simulink model "model"  (R2014a)
(part 3 of 4)

  bus249 : powerlib/Measurements/Load Flow Bus  LConnTagsString=a  ID=bus249  Vbase=110000  Vref=1  Vangle=0  VLF=1  angleLF=0
      settings: AttributesFormatString=|
      | %<ID>
      | %<Vbase>V
      | %<VLF>pu
      | %<angleLF>deg.
      | %<Name>
  bus25 : powerlib/Measurements/Load Flow Bus  LConnTagsString=a  ID=bus25  Vbase=110000  Vref=1  Vangle=0  VLF=1  angleLF=0
      settings: AttributesFormatString=|
      | %<ID>
      | %<Vbase>V
      | %<VLF>pu
      | %<angleLF>deg.
      | %<Name>
  bus250 : powerlib/Measurements/Load Flow Bus  LConnTagsString=a  ID=bus250  Vbase=110000  Vref=1  Vangle=0  VLF=1  angleLF=0
      settings: AttributesFormatString=|
      | %<ID>
      | %<Vbase>V
      | %<VLF>pu
      | %<angleLF>deg.
      | %<Name>
  bus251 : powerlib/Measurements/Load Flow Bus  LConnTagsString=a  ID=bus251  Vbase=110000  Vref=1  Vangle=0  VLF=1  angleLF=0
      settings: AttributesFormatString=|
      | %<ID>
      | %<Vbase>V
      | %<VLF>pu
      | %<angleLF>deg.
      | %<Name>
  bus252 : powerlib/Measurements/Load Flow Bus  LConnTagsString=a  ID=bus252  Vbase=110000  Vref=1  Vangle=0  VLF=1  angleLF=0
      settings: AttributesFormatString=|
      | %<ID>
      | %<Vbase>V
      | %<VLF>pu
      | %<angleLF>deg.
      | %<Name>
  bus253 : powerlib/Measurements/Load Flow Bus  LConnTagsString=a  ID=bus253  Vbase=110000  Vref=1  Vangle=0  VLF=1  angleLF=0
      settings: AttributesFormatString=|
      | %<ID>
      | %<Vbase>V
      | %<VLF>pu
      | %<angleLF>deg.
      | %<Name>
  bus254 : powerlib/Measurements/Load Flow Bus  LConnTagsString=a  ID=bus254  Vbase=110000  Vref=1  Vangle=0  VLF=1  angleLF=0
      settings: AttributesFormatString=|
      | %<ID>
      | %<Vbase>V
      | %<VLF>pu
      | %<angleLF>deg.
      | %<Name>
  bus255 : powerlib/Measurements/Load Flow Bus  LConnTagsString=a  ID=bus255  Vbase=110000  Vref=1  Vangle=0  VLF=1  angleLF=0
      settings: AttributesFormatString=|
      | %<ID>
      | %<Vbase>V
      | %<VLF>pu
      | %<angleLF>deg.
      | %<Name>
  bus256 : powerlib/Measurements/Load Flow Bus  LConnTagsString=a  ID=bus256  Vbase=110000  Vref=1  Vangle=0  VLF=1  angleLF=0
      settings: AttributesFormatString=|
      | %<ID>
      | %<Vbase>V
      | %<VLF>pu
      | %<angleLF>deg.
      | %<Name>
  bus257 : powerlib/Measurements/Load Flow Bus  LConnTagsString=a  ID=bus257  Vbase=110000  Vref=1  Vangle=0  VLF=1  angleLF=0
      settings: AttributesFormatString=|
      | %<ID>
      | %<Vbase>V
      | %<VLF>pu
      | %<angleLF>deg.
      | %<Name>
  bus258 : powerlib/Measurements/Load Flow Bus  LConnTagsString=a  ID=bus258  Vbase=110000  Vref=1  Vangle=0  VLF=1  angleLF=0
      settings: AttributesFormatString=|
      | %<ID>
      | %<Vbase>V
      | %<VLF>pu
      | %<angleLF>deg.
      | %<Name>
  bus259 : powerlib/Measurements/Load Flow Bus  LConnTagsString=a  ID=bus259  Vbase=110000  Vref=1  Vangle=0  VLF=1  angleLF=0
      settings: AttributesFormatString=|
      | %<ID>
      | %<Vbase>V
      | %<VLF>pu
      | %<angleLF>deg.
      | %<Name>
  bus26 : powerlib/Measurements/Load Flow Bus  LConnTagsString=a  ID=bus26  Vbase=110000  Vref=1  Vangle=0  VLF=1  angleLF=0
      settings: AttributesFormatString=|
      | %<ID>
      | %<Vbase>V
      | %<VLF>pu
      | %<angleLF>deg.
      | %<Name>
  bus260 : powerlib/Measurements/Load Flow Bus  LConnTagsString=a  ID=bus260  Vbase=110000  Vref=1  Vangle=0  VLF=1  angleLF=0
      settings: AttributesFormatString=|
      | %<ID>
      | %<Vbase>V
      | %<VLF>pu
      | %<angleLF>deg.
      | %<Name>
  bus261 : powerlib/Measurements/Load Flow Bus  LConnTagsString=a  ID=bus261  Vbase=110000  Vref=1  Vangle=0  VLF=1  angleLF=0
      settings: AttributesFormatString=|
      | %<ID>
      | %<Vbase>V
      | %<VLF>pu
      | %<angleLF>deg.
      | %<Name>
  bus262 : powerlib/Measurements/Load Flow Bus  LConnTagsString=a  ID=bus262  Vbase=110000  Vref=1  Vangle=0  VLF=1  angleLF=0
      settings: AttributesFormatString=|
      | %<ID>
      | %<Vbase>V
      | %<VLF>pu
      | %<angleLF>deg.
      | %<Name>
  bus263 : powerlib/Measurements/Load Flow Bus  LConnTagsString=a  ID=bus263  Vbase=110000  Vref=1  Vangle=0  VLF=1  angleLF=0
      settings: AttributesFormatString=|
      | %<ID>
      | %<Vbase>V
      | %<VLF>pu
      | %<angleLF>deg.
      | %<Name>
  bus264 : powerlib/Measurements/Load Flow Bus  LConnTagsString=a  ID=bus264  Vbase=110000  Vref=1  Vangle=0  VLF=1  angleLF=0
      settings: AttributesFormatString=|
      | %<ID>
      | %<Vbase>V
      | %<VLF>pu
      | %<angleLF>deg.
      | %<Name>
  bus265 : powerlib/Measurements/Load Flow Bus  LConnTagsString=a  ID=bus265  Vbase=110000  Vref=1  Vangle=0  VLF=1  angleLF=0
      settings: AttributesFormatString=|
      | %<ID>
      | %<Vbase>V
      | %<VLF>pu
      | %<angleLF>deg.
      | %<Name>
  bus266 : powerlib/Measurements/Load Flow Bus  LConnTagsString=a  ID=bus266  Vbase=110000  Vref=1  Vangle=0  VLF=1  angleLF=0
      settings: AttributesFormatString=|
      | %<ID>
      | %<Vbase>V
      | %<VLF>pu
      | %<angleLF>deg.
      | %<Name>
  bus267 : powerlib/Measurements/Load Flow Bus  LConnTagsString=a  ID=bus267  Vbase=110000  Vref=1  Vangle=0  VLF=1  angleLF=0
      settings: AttributesFormatString=|
      | %<ID>
      | %<Vbase>V
      | %<VLF>pu
      | %<angleLF>deg.
      | %<Name>
  bus268 : powerlib/Measurements/Load Flow Bus  LConnTagsString=a  ID=bus268  Vbase=110000  Vref=1  Vangle=0  VLF=1  angleLF=0
      settings: AttributesFormatString=|
      | %<ID>
      | %<Vbase>V
      | %<VLF>pu
      | %<angleLF>deg.
      | %<Name>
  bus269 : powerlib/Measurements/Load Flow Bus  LConnTagsString=a  ID=bus269  Vbase=110000  Vref=1  Vangle=0  VLF=1  angleLF=0
      settings: AttributesFormatString=|
      | %<ID>
      | %<Vbase>V
      | %<VLF>pu
      | %<angleLF>deg.
      | %<Name>
  bus27 : powerlib/Measurements/Load Flow Bus  LConnTagsString=a  ID=bus27  Vbase=110000  Vref=1  Vangle=0  VLF=1  angleLF=0
      settings: AttributesFormatString=|
      | %<ID>
      | %<Vbase>V
      | %<VLF>pu
      | %<angleLF>deg.
      | %<Name>
  bus270 : powerlib/Measurements/Load Flow Bus  LConnTagsString=a  ID=bus270  Vbase=110000  Vref=1  Vangle=0  VLF=1  angleLF=0
      settings: AttributesFormatString=|
      | %<ID>
      | %<Vbase>V
      | %<VLF>pu
      | %<angleLF>deg.
      | %<Name>
  bus271 : powerlib/Measurements/Load Flow Bus  LConnTagsString=a  ID=bus271  Vbase=110000  Vref=1  Vangle=0  VLF=1  angleLF=0
      settings: AttributesFormatString=|
      | %<ID>
      | %<Vbase>V
      | %<VLF>pu
      | %<angleLF>deg.
      | %<Name>
  bus272 : powerlib/Measurements/Load Flow Bus  LConnTagsString=a  ID=bus272  Vbase=110000  Vref=1  Vangle=0  VLF=1  angleLF=0
      settings: AttributesFormatString=|
      | %<ID>
      | %<Vbase>V
      | %<VLF>pu
      | %<angleLF>deg.
      | %<Name>
  bus273 : powerlib/Measurements/Load Flow Bus  LConnTagsString=a  ID=bus273  Vbase=110000  Vref=1  Vangle=0  VLF=1  angleLF=0
      settings: AttributesFormatString=|
      | %<ID>
      | %<Vbase>V
      | %<VLF>pu
      | %<angleLF>deg.
      | %<Name>
  bus274 : powerlib/Measurements/Load Flow Bus  LConnTagsString=a  ID=bus274  Vbase=110000  Vref=1  Vangle=0  VLF=1  angleLF=0
      settings: AttributesFormatString=|
      | %<ID>
      | %<Vbase>V
      | %<VLF>pu
      | %<angleLF>deg.
      | %<Name>
  bus275 : powerlib/Measurements/Load Flow Bus  LConnTagsString=a  ID=bus275  Vbase=110000  Vref=1  Vangle=0  VLF=1  angleLF=0
      settings: AttributesFormatString=|
      | %<ID>
      | %<Vbase>V
      | %<VLF>pu
      | %<angleLF>deg.
      | %<Name>
  bus276 : powerlib/Measurements/Load Flow Bus  LConnTagsString=a  ID=bus276  Vbase=110000  Vref=1  Vangle=0  VLF=1  angleLF=0
      settings: AttributesFormatString=|
      | %<ID>
      | %<Vbase>V
      | %<VLF>pu
      | %<angleLF>deg.
      | %<Name>
  bus277 : powerlib/Measurements/Load Flow Bus  LConnTagsString=a  ID=bus277  Vbase=110000  Vref=1  Vangle=0  VLF=1  angleLF=0
      settings: AttributesFormatString=|
      | %<ID>
      | %<Vbase>V
      | %<VLF>pu
      | %<angleLF>deg.
      | %<Name>
  bus278 : powerlib/Measurements/Load Flow Bus  LConnTagsString=a  ID=bus278  Vbase=110000  Vref=1  Vangle=0  VLF=1  angleLF=0
      settings: AttributesFormatString=|
      | %<ID>
      | %<Vbase>V
      | %<VLF>pu
      | %<angleLF>deg.
      | %<Name>
  bus279 : powerlib/Measurements/Load Flow Bus  LConnTagsString=a  ID=bus279  Vbase=110000  Vref=1  Vangle=0  VLF=1  angleLF=0
      settings: AttributesFormatString=|
      | %<ID>
      | %<Vbase>V
      | %<VLF>pu
      | %<angleLF>deg.
      | %<Name>
  bus28 : powerlib/Measurements/Load Flow Bus  LConnTagsString=a  ID=bus28  Vbase=110000  Vref=1  Vangle=0  VLF=1  angleLF=0
      settings: AttributesFormatString=|
      | %<ID>
      | %<Vbase>V
      | %<VLF>pu
      | %<angleLF>deg.
      | %<Name>
  bus280 : powerlib/Measurements/Load Flow Bus  LConnTagsString=a  ID=bus280  Vbase=110000  Vref=1  Vangle=0  VLF=1  angleLF=0
      settings: AttributesFormatString=|
      | %<ID>
      | %<Vbase>V
      | %<VLF>pu
      | %<angleLF>deg.
      | %<Name>
  bus281 : powerlib/Measurements/Load Flow Bus  LConnTagsString=a  ID=bus281  Vbase=110000  Vref=1  Vangle=0  VLF=1  angleLF=0
      settings: AttributesFormatString=|
      | %<ID>
      | %<Vbase>V
      | %<VLF>pu
      | %<angleLF>deg.
      | %<Name>
  bus282 : powerlib/Measurements/Load Flow Bus  LConnTagsString=a  ID=bus282  Vbase=110000  Vref=1  Vangle=0  VLF=1  angleLF=0
      settings: AttributesFormatString=|
      | %<ID>
      | %<Vbase>V
      | %<VLF>pu
      | %<angleLF>deg.
      | %<Name>
  bus283 : powerlib/Measurements/Load Flow Bus  LConnTagsString=a  ID=bus283  Vbase=110000  Vref=1  Vangle=0  VLF=1  angleLF=0
      settings: AttributesFormatString=|
      | %<ID>
      | %<Vbase>V
      | %<VLF>pu
      | %<angleLF>deg.
      | %<Name>
  bus284 : powerlib/Measurements/Load Flow Bus  LConnTagsString=a  ID=bus284  Vbase=110000  Vref=1  Vangle=0  VLF=1  angleLF=0
      settings: AttributesFormatString=|
      | %<ID>
      | %<Vbase>V
      | %<VLF>pu
      | %<angleLF>deg.
      | %<Name>
  bus285 : powerlib/Measurements/Load Flow Bus  LConnTagsString=a  ID=bus285  Vbase=110000  Vref=1  Vangle=0  VLF=1  angleLF=0
      settings: AttributesFormatString=|
      | %<ID>
      | %<Vbase>V
      | %<VLF>pu
      | %<angleLF>deg.
      | %<Name>
  bus286 : powerlib/Measurements/Load Flow Bus  LConnTagsString=a  ID=bus286  Vbase=110000  Vref=1  Vangle=0  VLF=1  angleLF=0
      settings: AttributesFormatString=|
      | %<ID>
      | %<Vbase>V
      | %<VLF>pu
      | %<angleLF>deg.
      | %<Name>
  bus287 : powerlib/Measurements/Load Flow Bus  LConnTagsString=a  ID=bus287  Vbase=110000  Vref=1  Vangle=0  VLF=1  angleLF=0
      settings: AttributesFormatString=|
      | %<ID>
      | %<Vbase>V
      | %<VLF>pu
      | %<angleLF>deg.
      | %<Name>
  bus288 : powerlib/Measurements/Load Flow Bus  LConnTagsString=a  ID=bus288  Vbase=110000  Vref=1  Vangle=0  VLF=1  angleLF=0
      settings: AttributesFormatString=|
      | %<ID>
      | %<Vbase>V
      | %<VLF>pu
      | %<angleLF>deg.
      | %<Name>
  bus289 : powerlib/Measurements/Load Flow Bus  LConnTagsString=a  ID=bus289  Vbase=110000  Vref=1  Vangle=0  VLF=1  angleLF=0
      settings: AttributesFormatString=|
      | %<ID>
      | %<Vbase>V
      | %<VLF>pu
      | %<angleLF>deg.
      | %<Name>
  bus29 : powerlib/Measurements/Load Flow Bus  LConnTagsString=a  ID=bus29  Vbase=110000  Vref=1  Vangle=0  VLF=1  angleLF=0
      settings: AttributesFormatString=|
      | %<ID>
      | %<Vbase>V
      | %<VLF>pu
      | %<angleLF>deg.
      | %<Name>
  bus290 : powerlib/Measurements/Load Flow Bus  LConnTagsString=a  ID=bus290  Vbase=110000  Vref=1  Vangle=0  VLF=1  angleLF=0
      settings: AttributesFormatString=|
      | %<ID>
      | %<Vbase>V
      | %<VLF>pu
      | %<angleLF>deg.
      | %<Name>
  bus291 : powerlib/Measurements/Load Flow Bus  LConnTagsString=a  ID=bus291  Vbase=110000  Vref=1  Vangle=0  VLF=1  angleLF=0
      settings: AttributesFormatString=|
      | %<ID>
      | %<Vbase>V
      | %<VLF>pu
      | %<angleLF>deg.
      | %<Name>
  bus292 : powerlib/Measurements/Load Flow Bus  LConnTagsString=a  ID=bus292  Vbase=110000  Vref=1  Vangle=0  VLF=1  angleLF=0
      settings: AttributesFormatString=|
      | %<ID>
      | %<Vbase>V
      | %<VLF>pu
      | %<angleLF>deg.
      | %<Name>
  bus293 : powerlib/Measurements/Load Flow Bus  LConnTagsString=a  ID=bus293  Vbase=110000  Vref=1  Vangle=0  VLF=1  angleLF=0
      settings: AttributesFormatString=|
      | %<ID>
      | %<Vbase>V
      | %<VLF>pu
      | %<angleLF>deg.
      | %<Name>
  bus294 : powerlib/Measurements/Load Flow Bus  LConnTagsString=a  ID=bus294  Vbase=110000  Vref=1  Vangle=0  VLF=1  angleLF=0
      settings: AttributesFormatString=|
      | %<ID>
      | %<Vbase>V
      | %<VLF>pu
      | %<angleLF>deg.
      | %<Name>
  bus295 : powerlib/Measurements/Load Flow Bus  LConnTagsString=a  ID=bus295  Vbase=110000  Vref=1  Vangle=0  VLF=1  angleLF=0
      settings: AttributesFormatString=|
      | %<ID>
      | %<Vbase>V
      | %<VLF>pu
      | %<angleLF>deg.
      | %<Name>
  bus296 : powerlib/Measurements/Load Flow Bus  LConnTagsString=a  ID=bus296  Vbase=110000  Vref=1  Vangle=0  VLF=1  angleLF=0
      settings: AttributesFormatString=|
      | %<ID>
      | %<Vbase>V
      | %<VLF>pu
      | %<angleLF>deg.
      | %<Name>
  bus297 : powerlib/Measurements/Load Flow Bus  LConnTagsString=a  ID=bus297  Vbase=110000  Vref=1  Vangle=0  VLF=1  angleLF=0
      settings: AttributesFormatString=|
      | %<ID>
      | %<Vbase>V
      | %<VLF>pu
      | %<angleLF>deg.
      | %<Name>
  bus298 : powerlib/Measurements/Load Flow Bus  LConnTagsString=a  ID=bus298  Vbase=110000  Vref=1  Vangle=0  VLF=1  angleLF=0
      settings: AttributesFormatString=|
      | %<ID>
      | %<Vbase>V
      | %<VLF>pu
      | %<angleLF>deg.
      | %<Name>
  bus299 : powerlib/Measurements/Load Flow Bus  LConnTagsString=a  ID=bus299  Vbase=110000  Vref=1  Vangle=0  VLF=1  angleLF=0
      settings: AttributesFormatString=|
      | %<ID>
      | %<Vbase>V
      | %<VLF>pu
      | %<angleLF>deg.
      | %<Name>
  bus3 : powerlib/Measurements/Load Flow Bus  LConnTagsString=a  ID=bus3  Vbase=110000  Vref=1  Vangle=0  VLF=1  angleLF=0
      settings: AttributesFormatString=|
      | %<ID>
      | %<Vbase>V
      | %<VLF>pu
      | %<angleLF>deg.
      | %<Name>
  bus30 : powerlib/Measurements/Load Flow Bus  LConnTagsString=a  ID=bus30  Vbase=110000  Vref=1  Vangle=0  VLF=1  angleLF=0
      settings: AttributesFormatString=|
      | %<ID>
      | %<Vbase>V
      | %<VLF>pu
      | %<angleLF>deg.
      | %<Name>
  bus300 : powerlib/Measurements/Load Flow Bus  LConnTagsString=a  ID=bus300  Vbase=110000  Vref=1  Vangle=0  VLF=1  angleLF=0
      settings: AttributesFormatString=|
      | %<ID>
      | %<Vbase>V
      | %<VLF>pu
      | %<angleLF>deg.
      | %<Name>
  bus301 : powerlib/Measurements/Load Flow Bus  LConnTagsString=a  ID=bus301  Vbase=110000  Vref=1  Vangle=0  VLF=1  angleLF=0
      settings: AttributesFormatString=|
      | %<ID>
      | %<Vbase>V
      | %<VLF>pu
      | %<angleLF>deg.
      | %<Name>
  bus302 : powerlib/Measurements/Load Flow Bus  LConnTagsString=a  ID=bus302  Vbase=110000  Vref=1  Vangle=0  VLF=1  angleLF=0
      settings: AttributesFormatString=|
      | %<ID>
      | %<Vbase>V
      | %<VLF>pu
      | %<angleLF>deg.
      | %<Name>
  bus303 : powerlib/Measurements/Load Flow Bus  LConnTagsString=a  ID=bus303  Vbase=110000  Vref=1  Vangle=0  VLF=1  angleLF=0
      settings: AttributesFormatString=|
      | %<ID>
      | %<Vbase>V
      | %<VLF>pu
      | %<angleLF>deg.
      | %<Name>
  bus304 : powerlib/Measurements/Load Flow Bus  LConnTagsString=a  ID=bus304  Vbase=110000  Vref=1  Vangle=0  VLF=1  angleLF=0
      settings: AttributesFormatString=|
      | %<ID>
      | %<Vbase>V
      | %<VLF>pu
      | %<angleLF>deg.
      | %<Name>
  bus305 : powerlib/Measurements/Load Flow Bus  LConnTagsString=a  ID=bus305  Vbase=110000  Vref=1  Vangle=0  VLF=1  angleLF=0
      settings: AttributesFormatString=|
      | %<ID>
      | %<Vbase>V
      | %<VLF>pu
      | %<angleLF>deg.
      | %<Name>
  bus306 : powerlib/Measurements/Load Flow Bus  LConnTagsString=a  ID=bus306  Vbase=110000  Vref=1  Vangle=0  VLF=1  angleLF=0
      settings: AttributesFormatString=|
      | %<ID>
      | %<Vbase>V
      | %<VLF>pu
      | %<angleLF>deg.
      | %<Name>
  bus307 : powerlib/Measurements/Load Flow Bus  LConnTagsString=a  ID=bus307  Vbase=110000  Vref=1  Vangle=0  VLF=1  angleLF=0
      settings: AttributesFormatString=|
      | %<ID>
      | %<Vbase>V
      | %<VLF>pu
      | %<angleLF>deg.
      | %<Name>
  bus308 : powerlib/Measurements/Load Flow Bus  LConnTagsString=a  ID=bus308  Vbase=110000  Vref=1  Vangle=0  VLF=1  angleLF=0
      settings: AttributesFormatString=|
      | %<ID>
      | %<Vbase>V
      | %<VLF>pu
      | %<angleLF>deg.
      | %<Name>
  bus309 : powerlib/Measurements/Load Flow Bus  LConnTagsString=a  ID=bus309  Vbase=110000  Vref=1  Vangle=0  VLF=1  angleLF=0
      settings: AttributesFormatString=|
      | %<ID>
      | %<Vbase>V
      | %<VLF>pu
      | %<angleLF>deg.
      | %<Name>
  bus31 : powerlib/Measurements/Load Flow Bus  LConnTagsString=a  ID=bus31  Vbase=110000  Vref=1  Vangle=0  VLF=1  angleLF=0
      settings: AttributesFormatString=|
      | %<ID>
      | %<Vbase>V
      | %<VLF>pu
      | %<angleLF>deg.
      | %<Name>
  bus310 : powerlib/Measurements/Load Flow Bus  LConnTagsString=a  ID=bus310  Vbase=110000  Vref=1  Vangle=0  VLF=1  angleLF=0
      settings: AttributesFormatString=|
      | %<ID>
      | %<Vbase>V
      | %<VLF>pu
      | %<angleLF>deg.
      | %<Name>
  bus311 : powerlib/Measurements/Load Flow Bus  LConnTagsString=a  ID=bus311  Vbase=110000  Vref=1  Vangle=0  VLF=1  angleLF=0
      settings: AttributesFormatString=|
      | %<ID>
      | %<Vbase>V
      | %<VLF>pu
      | %<angleLF>deg.
      | %<Name>
  bus312 : powerlib/Measurements/Load Flow Bus  LConnTagsString=a  ID=bus312  Vbase=110000  Vref=1  Vangle=0  VLF=1  angleLF=0
      settings: AttributesFormatString=|
      | %<ID>
      | %<Vbase>V
      | %<VLF>pu
      | %<angleLF>deg.
      | %<Name>
  bus313 : powerlib/Measurements/Load Flow Bus  LConnTagsString=a  ID=bus313  Vbase=110000  Vref=1  Vangle=0  VLF=1  angleLF=0
      settings: AttributesFormatString=|
      | %<ID>
      | %<Vbase>V
      | %<VLF>pu
      | %<angleLF>deg.
      | %<Name>
  bus314 : powerlib/Measurements/Load Flow Bus  LConnTagsString=a  ID=bus314  Vbase=110000  Vref=1  Vangle=0  VLF=1  angleLF=0
      settings: AttributesFormatString=|
      | %<ID>
      | %<Vbase>V
      | %<VLF>pu
      | %<angleLF>deg.
      | %<Name>
  bus315 : powerlib/Measurements/Load Flow Bus  LConnTagsString=a  ID=bus315  Vbase=110000  Vref=1  Vangle=0  VLF=1  angleLF=0
      settings: AttributesFormatString=|
      | %<ID>
      | %<Vbase>V
      | %<VLF>pu
      | %<angleLF>deg.
      | %<Name>
  bus316 : powerlib/Measurements/Load Flow Bus  LConnTagsString=a  ID=bus316  Vbase=110000  Vref=1  Vangle=0  VLF=1  angleLF=0
      settings: AttributesFormatString=|
      | %<ID>
      | %<Vbase>V
      | %<VLF>pu
      | %<angleLF>deg.
      | %<Name>
  bus317 : powerlib/Measurements/Load Flow Bus  LConnTagsString=a  ID=bus317  Vbase=110000  Vref=1  Vangle=0  VLF=1  angleLF=0
      settings: AttributesFormatString=|
      | %<ID>
      | %<Vbase>V
      | %<VLF>pu
      | %<angleLF>deg.
      | %<Name>
  bus318 : powerlib/Measurements/Load Flow Bus  LConnTagsString=a  ID=bus318  Vbase=110000  Vref=1  Vangle=0  VLF=1  angleLF=0
      settings: AttributesFormatString=|
      | %<ID>
      | %<Vbase>V
      | %<VLF>pu
      | %<angleLF>deg.
      | %<Name>
  bus319 : powerlib/Measurements/Load Flow Bus  LConnTagsString=a  ID=bus319  Vbase=110000  Vref=1  Vangle=0  VLF=1  angleLF=0
      settings: AttributesFormatString=|
      | %<ID>
      | %<Vbase>V
      | %<VLF>pu
      | %<angleLF>deg.
      | %<Name>
  bus32 : powerlib/Measurements/Load Flow Bus  LConnTagsString=a  ID=bus32  Vbase=110000  Vref=1  Vangle=0  VLF=1  angleLF=0
      settings: AttributesFormatString=|
      | %<ID>
      | %<Vbase>V
      | %<VLF>pu
      | %<angleLF>deg.
      | %<Name>
  bus320 : powerlib/Measurements/Load Flow Bus  LConnTagsString=a  ID=bus320  Vbase=110000  Vref=1  Vangle=0  VLF=1  angleLF=0
      settings: AttributesFormatString=|
      | %<ID>
      | %<Vbase>V
      | %<VLF>pu
      | %<angleLF>deg.
      | %<Name>
  bus321 : powerlib/Measurements/Load Flow Bus  LConnTagsString=a  ID=bus321  Vbase=110000  Vref=1  Vangle=0  VLF=1  angleLF=0
      settings: AttributesFormatString=|
      | %<ID>
      | %<Vbase>V
      | %<VLF>pu
      | %<angleLF>deg.
      | %<Name>
  bus322 : powerlib/Measurements/Load Flow Bus  LConnTagsString=a  ID=bus322  Vbase=110000  Vref=1  Vangle=0  VLF=1  angleLF=0
      settings: AttributesFormatString=|
      | %<ID>
      | %<Vbase>V
      | %<VLF>pu
      | %<angleLF>deg.
      | %<Name>
  bus323 : powerlib/Measurements/Load Flow Bus  LConnTagsString=a  ID=bus323  Vbase=110000  Vref=1  Vangle=0  VLF=1  angleLF=0
      settings: AttributesFormatString=|
      | %<ID>
      | %<Vbase>V
      | %<VLF>pu
      | %<angleLF>deg.
      | %<Name>
  bus324 : powerlib/Measurements/Load Flow Bus  LConnTagsString=a  ID=bus324  Vbase=110000  Vref=1  Vangle=0  VLF=1  angleLF=0
      settings: AttributesFormatString=|
      | %<ID>
      | %<Vbase>V
      | %<VLF>pu
      | %<angleLF>deg.
      | %<Name>
  bus325 : powerlib/Measurements/Load Flow Bus  LConnTagsString=a  ID=bus325  Vbase=110000  Vref=1  Vangle=0  VLF=1  angleLF=0
      settings: AttributesFormatString=|
      | %<ID>
      | %<Vbase>V
      | %<VLF>pu
      | %<angleLF>deg.
      | %<Name>
  bus326 : powerlib/Measurements/Load Flow Bus  LConnTagsString=a  ID=bus326  Vbase=110000  Vref=1  Vangle=0  VLF=1  angleLF=0
      settings: AttributesFormatString=|
      | %<ID>
      | %<Vbase>V
      | %<VLF>pu
      | %<angleLF>deg.
      | %<Name>
  bus327 : powerlib/Measurements/Load Flow Bus  LConnTagsString=a  ID=bus327  Vbase=110000  Vref=1  Vangle=0  VLF=1  angleLF=0
      settings: AttributesFormatString=|
      | %<ID>
      | %<Vbase>V
      | %<VLF>pu
      | %<angleLF>deg.
      | %<Name>
  bus328 : powerlib/Measurements/Load Flow Bus  LConnTagsString=a  ID=bus328  Vbase=110000  Vref=1  Vangle=0  VLF=1  angleLF=0
      settings: AttributesFormatString=|
      | %<ID>
      | %<Vbase>V
      | %<VLF>pu
      | %<angleLF>deg.
      | %<Name>
  bus329 : powerlib/Measurements/Load Flow Bus  LConnTagsString=a  ID=bus329  Vbase=110000  Vref=1  Vangle=0  VLF=1  angleLF=0
      settings: AttributesFormatString=|
      | %<ID>
      | %<Vbase>V
      | %<VLF>pu
      | %<angleLF>deg.
      | %<Name>
  bus33 : powerlib/Measurements/Load Flow Bus  LConnTagsString=a  ID=bus33  Vbase=110000  Vref=1  Vangle=0  VLF=1  angleLF=0
      settings: AttributesFormatString=|
      | %<ID>
      | %<Vbase>V
      | %<VLF>pu
      | %<angleLF>deg.
      | %<Name>
  bus330 : powerlib/Measurements/Load Flow Bus  LConnTagsString=a  ID=bus330  Vbase=110000  Vref=1  Vangle=0  VLF=1  angleLF=0
      settings: AttributesFormatString=|
      | %<ID>
      | %<Vbase>V
      | %<VLF>pu
      | %<angleLF>deg.
      | %<Name>
  bus331 : powerlib/Measurements/Load Flow Bus  LConnTagsString=a  ID=bus331  Vbase=110000  Vref=1  Vangle=0  VLF=1  angleLF=0
      settings: AttributesFormatString=|
      | %<ID>
      | %<Vbase>V
      | %<VLF>pu
      | %<angleLF>deg.
      | %<Name>
  bus332 : powerlib/Measurements/Load Flow Bus  LConnTagsString=a  ID=bus332  Vbase=110000  Vref=1  Vangle=0  VLF=1  angleLF=0
      settings: AttributesFormatString=|
      | %<ID>
      | %<Vbase>V
      | %<VLF>pu
      | %<angleLF>deg.
      | %<Name>
  bus333 : powerlib/Measurements/Load Flow Bus  LConnTagsString=a  ID=bus333  Vbase=110000  Vref=1  Vangle=0  VLF=1  angleLF=0
      settings: AttributesFormatString=|
      | %<ID>
      | %<Vbase>V
      | %<VLF>pu
      | %<angleLF>deg.
      | %<Name>
  bus334 : powerlib/Measurements/Load Flow Bus  LConnTagsString=a  ID=bus334  Vbase=110000  Vref=1  Vangle=0  VLF=1  angleLF=0
      settings: AttributesFormatString=|
      | %<ID>
      | %<Vbase>V
      | %<VLF>pu
      | %<angleLF>deg.
      | %<Name>
  bus335 : powerlib/Measurements/Load Flow Bus  LConnTagsString=a  ID=bus335  Vbase=110000  Vref=1  Vangle=0  VLF=1  angleLF=0
      settings: AttributesFormatString=|
      | %<ID>
      | %<Vbase>V
      | %<VLF>pu
      | %<angleLF>deg.
      | %<Name>
  bus336 : powerlib/Measurements/Load Flow Bus  LConnTagsString=a  ID=bus336  Vbase=110000  Vref=1  Vangle=0  VLF=1  angleLF=0
      settings: AttributesFormatString=|
      | %<ID>
      | %<Vbase>V
      | %<VLF>pu
      | %<angleLF>deg.
      | %<Name>
  bus337 : powerlib/Measurements/Load Flow Bus  LConnTagsString=a  ID=bus337  Vbase=110000  Vref=1  Vangle=0  VLF=1  angleLF=0
      settings: AttributesFormatString=|
      | %<ID>
      | %<Vbase>V
      | %<VLF>pu
      | %<angleLF>deg.
      | %<Name>
  bus338 : powerlib/Measurements/Load Flow Bus  LConnTagsString=a  ID=bus338  Vbase=110000  Vref=1  Vangle=0  VLF=1  angleLF=0
      settings: AttributesFormatString=|
      | %<ID>
      | %<Vbase>V
      | %<VLF>pu
      | %<angleLF>deg.
      | %<Name>
  bus339 : powerlib/Measurements/Load Flow Bus  LConnTagsString=a  ID=bus339  Vbase=110000  Vref=1  Vangle=0  VLF=1  angleLF=0
      settings: AttributesFormatString=|
      | %<ID>
      | %<Vbase>V
      | %<VLF>pu
      | %<angleLF>deg.
      | %<Name>
  bus34 : powerlib/Measurements/Load Flow Bus  LConnTagsString=a  ID=bus34  Vbase=110000  Vref=1  Vangle=0  VLF=1  angleLF=0
      settings: AttributesFormatString=|
      | %<ID>
      | %<Vbase>V
      | %<VLF>pu
      | %<angleLF>deg.
      | %<Name>
  bus340 : powerlib/Measurements/Load Flow Bus  LConnTagsString=a  ID=bus340  Vbase=110000  Vref=1  Vangle=0  VLF=1  angleLF=0
      settings: AttributesFormatString=|
      | %<ID>
      | %<Vbase>V
      | %<VLF>pu
      | %<angleLF>deg.
      | %<Name>
  bus341 : powerlib/Measurements/Load Flow Bus  LConnTagsString=a  ID=bus341  Vbase=110000  Vref=1  Vangle=0  VLF=1  angleLF=0
      settings: AttributesFormatString=|
      | %<ID>
      | %<Vbase>V
      | %<VLF>pu
      | %<angleLF>deg.
      | %<Name>
  bus342 : powerlib/Measurements/Load Flow Bus  LConnTagsString=a  ID=bus342  Vbase=110000  Vref=1  Vangle=0  VLF=1  angleLF=0
      settings: AttributesFormatString=|
      | %<ID>
      | %<Vbase>V
      | %<VLF>pu
      | %<angleLF>deg.
      | %<Name>
  bus343 : powerlib/Measurements/Load Flow Bus  LConnTagsString=a  ID=bus343  Vbase=110000  Vref=1  Vangle=0  VLF=1  angleLF=0
      settings: AttributesFormatString=|
      | %<ID>
      | %<Vbase>V
      | %<VLF>pu
      | %<angleLF>deg.
      | %<Name>
  bus344 : powerlib/Measurements/Load Flow Bus  LConnTagsString=a  ID=bus344  Vbase=110000  Vref=1  Vangle=0  VLF=1  angleLF=0
      settings: AttributesFormatString=|
      | %<ID>
      | %<Vbase>V
      | %<VLF>pu
      | %<angleLF>deg.
      | %<Name>
  bus345 : powerlib/Measurements/Load Flow Bus  LConnTagsString=a  ID=bus345  Vbase=110000  Vref=1  Vangle=0  VLF=1  angleLF=0
      settings: AttributesFormatString=|
      | %<ID>
      | %<Vbase>V
      | %<VLF>pu
      | %<angleLF>deg.
      | %<Name>
  bus346 : powerlib/Measurements/Load Flow Bus  LConnTagsString=a  ID=bus346  Vbase=110000  Vref=1  Vangle=0  VLF=1  angleLF=0
      settings: AttributesFormatString=|
      | %<ID>
      | %<Vbase>V
      | %<VLF>pu
      | %<angleLF>deg.
      | %<Name>
  bus347 : powerlib/Measurements/Load Flow Bus  LConnTagsString=a  ID=bus347  Vbase=110000  Vref=1  Vangle=0  VLF=1  angleLF=0
      settings: AttributesFormatString=|
      | %<ID>
      | %<Vbase>V
      | %<VLF>pu
      | %<angleLF>deg.
      | %<Name>
  bus348 : powerlib/Measurements/Load Flow Bus  LConnTagsString=a  ID=bus348  Vbase=110000  Vref=1  Vangle=0  VLF=1  angleLF=0
      settings: AttributesFormatString=|
      | %<ID>
      | %<Vbase>V
      | %<VLF>pu
      | %<angleLF>deg.
      | %<Name>
  bus349 : powerlib/Measurements/Load Flow Bus  LConnTagsString=a  ID=bus349  Vbase=110000  Vref=1  Vangle=0  VLF=1  angleLF=0
      settings: AttributesFormatString=|
      | %<ID>
      | %<Vbase>V
      | %<VLF>pu
      | %<angleLF>deg.
      | %<Name>
  bus35 : powerlib/Measurements/Load Flow Bus  LConnTagsString=a  ID=bus35  Vbase=110000  Vref=1  Vangle=0  VLF=1  angleLF=0
      settings: AttributesFormatString=|
      | %<ID>
      | %<Vbase>V
      | %<VLF>pu
      | %<angleLF>deg.
      | %<Name>
  bus350 : powerlib/Measurements/Load Flow Bus  LConnTagsString=a  ID=bus350  Vbase=110000  Vref=1  Vangle=0  VLF=1  angleLF=0
      settings: AttributesFormatString=|
      | %<ID>
      | %<Vbase>V
      | %<VLF>pu
      | %<angleLF>deg.
      | %<Name>
  bus351 : powerlib/Measurements/Load Flow Bus  LConnTagsString=a  ID=bus351  Vbase=110000  Vref=1  Vangle=0  VLF=1  angleLF=0
      settings: AttributesFormatString=|
      | %<ID>
      | %<Vbase>V
      | %<VLF>pu
      | %<angleLF>deg.
      | %<Name>
  bus352 : powerlib/Measurements/Load Flow Bus  LConnTagsString=a  ID=bus352  Vbase=110000  Vref=1  Vangle=0  VLF=1  angleLF=0
      settings: AttributesFormatString=|
      | %<ID>
      | %<Vbase>V
      | %<VLF>pu
      | %<angleLF>deg.
      | %<Name>
  bus353 : powerlib/Measurements/Load Flow Bus  LConnTagsString=a  ID=bus353  Vbase=110000  Vref=1  Vangle=0  VLF=1  angleLF=0
      settings: AttributesFormatString=|
      | %<ID>
      | %<Vbase>V
      | %<VLF>pu
      | %<angleLF>deg.
      | %<Name>
  bus354 : powerlib/Measurements/Load Flow Bus  LConnTagsString=a  ID=bus354  Vbase=110000  Vref=1  Vangle=0  VLF=1  angleLF=0
      settings: AttributesFormatString=|
      | %<ID>
      | %<Vbase>V
      | %<VLF>pu
      | %<angleLF>deg.
      | %<Name>
  bus355 : powerlib/Measurements/Load Flow Bus  LConnTagsString=a  ID=bus355  Vbase=110000  Vref=1  Vangle=0  VLF=1  angleLF=0
      settings: AttributesFormatString=|
      | %<ID>
      | %<Vbase>V
      | %<VLF>pu
      | %<angleLF>deg.
      | %<Name>
  bus356 : powerlib/Measurements/Load Flow Bus  LConnTagsString=a  ID=bus356  Vbase=110000  Vref=1  Vangle=0  VLF=1  angleLF=0
      settings: AttributesFormatString=|
      | %<ID>
      | %<Vbase>V
      | %<VLF>pu
      | %<angleLF>deg.
      | %<Name>
  bus357 : powerlib/Measurements/Load Flow Bus  LConnTagsString=a  ID=bus357  Vbase=110000  Vref=1  Vangle=0  VLF=1  angleLF=0
      settings: AttributesFormatString=|
      | %<ID>
      | %<Vbase>V
      | %<VLF>pu
      | %<angleLF>deg.
      | %<Name>
  bus358 : powerlib/Measurements/Load Flow Bus  LConnTagsString=a  ID=bus358  Vbase=110000  Vref=1  Vangle=0  VLF=1  angleLF=0
      settings: AttributesFormatString=|
      | %<ID>
      | %<Vbase>V
      | %<VLF>pu
      | %<angleLF>deg.
      | %<Name>
  bus359 : powerlib/Measurements/Load Flow Bus  LConnTagsString=a  ID=bus359  Vbase=110000  Vref=1  Vangle=0  VLF=1  angleLF=0
      settings: AttributesFormatString=|
      | %<ID>
      | %<Vbase>V
      | %<VLF>pu
      | %<angleLF>deg.
      | %<Name>
  bus36 : powerlib/Measurements/Load Flow Bus  LConnTagsString=a  ID=bus36  Vbase=110000  Vref=1  Vangle=0  VLF=1  angleLF=0
      settings: AttributesFormatString=|
      | %<ID>
      | %<Vbase>V
      | %<VLF>pu
      | %<angleLF>deg.
      | %<Name>
  bus360 : powerlib/Measurements/Load Flow Bus  LConnTagsString=a  ID=bus360  Vbase=110000  Vref=1  Vangle=0  VLF=1  angleLF=0
      settings: AttributesFormatString=|
      | %<ID>
      | %<Vbase>V
      | %<VLF>pu
      | %<angleLF>deg.
      | %<Name>
  bus361 : powerlib/Measurements/Load Flow Bus  LConnTagsString=a  ID=bus361  Vbase=110000  Vref=1  Vangle=0  VLF=1  angleLF=0
      settings: AttributesFormatString=|
      | %<ID>
      | %<Vbase>V
      | %<VLF>pu
      | %<angleLF>deg.
      | %<Name>
  bus362 : powerlib/Measurements/Load Flow Bus  LConnTagsString=a  ID=bus362  Vbase=110000  Vref=1  Vangle=0  VLF=1  angleLF=0
      settings: AttributesFormatString=|
      | %<ID>
      | %<Vbase>V
      | %<VLF>pu
      | %<angleLF>deg.
      | %<Name>
  bus363 : powerlib/Measurements/Load Flow Bus  LConnTagsString=a  ID=bus363  Vbase=110000  Vref=1  Vangle=0  VLF=1  angleLF=0
      settings: AttributesFormatString=|
      | %<ID>
      | %<Vbase>V
      | %<VLF>pu
      | %<angleLF>deg.
      | %<Name>
  bus364 : powerlib/Measurements/Load Flow Bus  LConnTagsString=a  ID=bus364  Vbase=110000  Vref=1  Vangle=0  VLF=1  angleLF=0
      settings: AttributesFormatString=|
      | %<ID>
      | %<Vbase>V
      | %<VLF>pu
      | %<angleLF>deg.
      | %<Name>
  bus365 : powerlib/Measurements/Load Flow Bus  LConnTagsString=a  ID=bus365  Vbase=110000  Vref=1  Vangle=0  VLF=1  angleLF=0
      settings: AttributesFormatString=|
      | %<ID>
      | %<Vbase>V
      | %<VLF>pu
      | %<angleLF>deg.
      | %<Name>
  bus366 : powerlib/Measurements/Load Flow Bus  LConnTagsString=a  ID=bus366  Vbase=110000  Vref=1  Vangle=0  VLF=1  angleLF=0
      settings: AttributesFormatString=|
      | %<ID>
      | %<Vbase>V
      | %<VLF>pu
      | %<angleLF>deg.
      | %<Name>
  bus367 : powerlib/Measurements/Load Flow Bus  LConnTagsString=a  ID=bus367  Vbase=110000  Vref=1  Vangle=0  VLF=1  angleLF=0
      settings: AttributesFormatString=|
      | %<ID>
      | %<Vbase>V
      | %<VLF>pu
      | %<angleLF>deg.
      | %<Name>
  bus368 : powerlib/Measurements/Load Flow Bus  LConnTagsString=a  ID=bus368  Vbase=110000  Vref=1  Vangle=0  VLF=1  angleLF=0
      settings: AttributesFormatString=|
      | %<ID>
      | %<Vbase>V
      | %<VLF>pu
      | %<angleLF>deg.
      | %<Name>
  bus369 : powerlib/Measurements/Load Flow Bus  LConnTagsString=a  ID=bus369  Vbase=110000  Vref=1  Vangle=0  VLF=1  angleLF=0
      settings: AttributesFormatString=|
      | %<ID>
      | %<Vbase>V
      | %<VLF>pu
      | %<angleLF>deg.
      | %<Name>
  bus37 : powerlib/Measurements/Load Flow Bus  LConnTagsString=a  ID=bus37  Vbase=110000  Vref=1  Vangle=0  VLF=1  angleLF=0
      settings: AttributesFormatString=|
      | %<ID>
      | %<Vbase>V
      | %<VLF>pu
      | %<angleLF>deg.
      | %<Name>
  bus370 : powerlib/Measurements/Load Flow Bus  LConnTagsString=a  ID=bus370  Vbase=110000  Vref=1  Vangle=0  VLF=1  angleLF=0
      settings: AttributesFormatString=|
      | %<ID>
      | %<Vbase>V
      | %<VLF>pu
      | %<angleLF>deg.
      | %<Name>
  bus371 : powerlib/Measurements/Load Flow Bus  LConnTagsString=a  ID=bus371  Vbase=110000  Vref=1  Vangle=0  VLF=1  angleLF=0
      settings: AttributesFormatString=|
      | %<ID>
      | %<Vbase>V
      | %<VLF>pu
      | %<angleLF>deg.
      | %<Name>
  bus372 : powerlib/Measurements/Load Flow Bus  LConnTagsString=a  ID=bus372  Vbase=330000  Vref=1  Vangle=0  VLF=1  angleLF=0
      settings: AttributesFormatString=|
      | %<ID>
      | %<Vbase>V
      | %<VLF>pu
      | %<angleLF>deg.
      | %<Name>
  bus373 : powerlib/Measurements/Load Flow Bus  LConnTagsString=a  ID=bus373  Vbase=330000  Vref=1  Vangle=0  VLF=1  angleLF=0
      settings: AttributesFormatString=|
      | %<ID>
      | %<Vbase>V
      | %<VLF>pu
      | %<angleLF>deg.
      | %<Name>
  bus374 : powerlib/Measurements/Load Flow Bus  LConnTagsString=a  ID=bus374  Vbase=330000  Vref=1  Vangle=0  VLF=1  angleLF=0
      settings: AttributesFormatString=|
      | %<ID>
      | %<Vbase>V
      | %<VLF>pu
      | %<angleLF>deg.
      | %<Name>
  bus375 : powerlib/Measurements/Load Flow Bus  LConnTagsString=a  ID=bus375  Vbase=330000  Vref=1  Vangle=0  VLF=1  angleLF=0
      settings: AttributesFormatString=|
      | %<ID>
      | %<Vbase>V
      | %<VLF>pu
      | %<angleLF>deg.
      | %<Name>
  bus376 : powerlib/Measurements/Load Flow Bus  LConnTagsString=a  ID=bus376  Vbase=330000  Vref=1  Vangle=0  VLF=1  angleLF=0
      settings: AttributesFormatString=|
      | %<ID>
      | %<Vbase>V
      | %<VLF>pu
      | %<angleLF>deg.
      | %<Name>
  bus38 : powerlib/Measurements/Load Flow Bus  LConnTagsString=a  ID=bus38  Vbase=110000  Vref=1  Vangle=0  VLF=1  angleLF=0
      settings: AttributesFormatString=|
      | %<ID>
      | %<Vbase>V
      | %<VLF>pu
      | %<angleLF>deg.
      | %<Name>
  bus39 : powerlib/Measurements/Load Flow Bus  LConnTagsString=a  ID=bus39  Vbase=110000  Vref=1  Vangle=0  VLF=1  angleLF=0
      settings: AttributesFormatString=|
      | %<ID>
      | %<Vbase>V
      | %<VLF>pu
      | %<angleLF>deg.
      | %<Name>
  bus4 : powerlib/Measurements/Load Flow Bus  LConnTagsString=a  ID=bus4  Vbase=110000  Vref=1  Vangle=0  VLF=1  angleLF=0
      settings: AttributesFormatString=|
      | %<ID>
      | %<Vbase>V
      | %<VLF>pu
      | %<angleLF>deg.
      | %<Name>
  bus40 : powerlib/Measurements/Load Flow Bus  LConnTagsString=a  ID=bus40  Vbase=110000  Vref=1  Vangle=0  VLF=1  angleLF=0
      settings: AttributesFormatString=|
      | %<ID>
      | %<Vbase>V
      | %<VLF>pu
      | %<angleLF>deg.
      | %<Name>
  bus41 : powerlib/Measurements/Load Flow Bus  LConnTagsString=a  ID=bus41  Vbase=110000  Vref=1  Vangle=0  VLF=1  angleLF=0
      settings: AttributesFormatString=|
      | %<ID>
      | %<Vbase>V
      | %<VLF>pu
      | %<angleLF>deg.
      | %<Name>
  bus42 : powerlib/Measurements/Load Flow Bus  LConnTagsString=a  ID=bus42  Vbase=110000  Vref=1  Vangle=0  VLF=1  angleLF=0
      settings: AttributesFormatString=|
      | %<ID>
      | %<Vbase>V
      | %<VLF>pu
      | %<angleLF>deg.
      | %<Name>
  bus43 : powerlib/Measurements/Load Flow Bus  LConnTagsString=a  ID=bus43  Vbase=110000  Vref=1  Vangle=0  VLF=1  angleLF=0
      settings: AttributesFormatString=|
      | %<ID>
      | %<Vbase>V
      | %<VLF>pu
      | %<angleLF>deg.
      | %<Name>
  bus44 : powerlib/Measurements/Load Flow Bus  LConnTagsString=a  ID=bus44  Vbase=110000  Vref=1  Vangle=0  VLF=1  angleLF=0
      settings: AttributesFormatString=|
      | %<ID>
      | %<Vbase>V
      | %<VLF>pu
      | %<angleLF>deg.
      | %<Name>
  bus45 : powerlib/Measurements/Load Flow Bus  LConnTagsString=a  ID=bus45  Vbase=110000  Vref=1  Vangle=0  VLF=1  angleLF=0
      settings: AttributesFormatString=|
      | %<ID>
      | %<Vbase>V
      | %<VLF>pu
      | %<angleLF>deg.
      | %<Name>
  bus46 : powerlib/Measurements/Load Flow Bus  LConnTagsString=a  ID=bus46  Vbase=110000  Vref=1  Vangle=0  VLF=1  angleLF=0
      settings: AttributesFormatString=|
      | %<ID>
      | %<Vbase>V
      | %<VLF>pu
      | %<angleLF>deg.
      | %<Name>
  bus47 : powerlib/Measurements/Load Flow Bus  LConnTagsString=a  ID=bus47  Vbase=110000  Vref=1  Vangle=0  VLF=1  angleLF=0
      settings: AttributesFormatString=|
      | %<ID>
      | %<Vbase>V
      | %<VLF>pu
      | %<angleLF>deg.
      | %<Name>
  bus48 : powerlib/Measurements/Load Flow Bus  LConnTagsString=a  ID=bus48  Vbase=110000  Vref=1  Vangle=0  VLF=1  angleLF=0
      settings: AttributesFormatString=|
      | %<ID>
      | %<Vbase>V
      | %<VLF>pu
      | %<angleLF>deg.
      | %<Name>
  bus49 : powerlib/Measurements/Load Flow Bus  LConnTagsString=a  ID=bus49  Vbase=110000  Vref=1  Vangle=0  VLF=1  angleLF=0
      settings: AttributesFormatString=|
      | %<ID>
      | %<Vbase>V
      | %<VLF>pu
      | %<angleLF>deg.
      | %<Name>
  bus5 : powerlib/Measurements/Load Flow Bus  LConnTagsString=a  ID=bus5  Vbase=110000  Vref=1  Vangle=0  VLF=1  angleLF=0
      settings: AttributesFormatString=|
      | %<ID>
      | %<Vbase>V
      | %<VLF>pu
      | %<angleLF>deg.
      | %<Name>
  bus50 : powerlib/Measurements/Load Flow Bus  LConnTagsString=a  ID=bus50  Vbase=110000  Vref=1  Vangle=0  VLF=1  angleLF=0
      settings: AttributesFormatString=|
      | %<ID>
      | %<Vbase>V
      | %<VLF>pu
      | %<angleLF>deg.
      | %<Name>
  bus51 : powerlib/Measurements/Load Flow Bus  LConnTagsString=a  ID=bus51  Vbase=110000  Vref=1  Vangle=0  VLF=1  angleLF=0
      settings: AttributesFormatString=|
      | %<ID>
      | %<Vbase>V
      | %<VLF>pu
      | %<angleLF>deg.
      | %<Name>
  bus52 : powerlib/Measurements/Load Flow Bus  LConnTagsString=a  ID=bus52  Vbase=110000  Vref=1  Vangle=0  VLF=1  angleLF=0
      settings: AttributesFormatString=|
      | %<ID>
      | %<Vbase>V
      | %<VLF>pu
      | %<angleLF>deg.
      | %<Name>
  bus53 : powerlib/Measurements/Load Flow Bus  LConnTagsString=a  ID=bus53  Vbase=110000  Vref=1  Vangle=0  VLF=1  angleLF=0
      settings: AttributesFormatString=|
      | %<ID>
      | %<Vbase>V
      | %<VLF>pu
      | %<angleLF>deg.
      | %<Name>
  bus54 : powerlib/Measurements/Load Flow Bus  LConnTagsString=a  ID=bus54  Vbase=110000  Vref=1  Vangle=0  VLF=1  angleLF=0
      settings: AttributesFormatString=|
      | %<ID>
      | %<Vbase>V
      | %<VLF>pu
      | %<angleLF>deg.
      | %<Name>
  bus55 : powerlib/Measurements/Load Flow Bus  LConnTagsString=a  ID=bus55  Vbase=110000  Vref=1  Vangle=0  VLF=1  angleLF=0
      settings: AttributesFormatString=|
      | %<ID>
      | %<Vbase>V
      | %<VLF>pu
      | %<angleLF>deg.
      | %<Name>
  bus56 : powerlib/Measurements/Load Flow Bus  LConnTagsString=a  ID=bus56  Vbase=110000  Vref=1  Vangle=0  VLF=1  angleLF=0
      settings: AttributesFormatString=|
      | %<ID>
      | %<Vbase>V
      | %<VLF>pu
      | %<angleLF>deg.
      | %<Name>
  bus57 : powerlib/Measurements/Load Flow Bus  LConnTagsString=a  ID=bus57  Vbase=110000  Vref=1  Vangle=0  VLF=1  angleLF=0
      settings: AttributesFormatString=|
      | %<ID>
      | %<Vbase>V
      | %<VLF>pu
      | %<angleLF>deg.
      | %<Name>
  bus58 : powerlib/Measurements/Load Flow Bus  LConnTagsString=a  ID=bus58  Vbase=110000  Vref=1  Vangle=0  VLF=1  angleLF=0
      settings: AttributesFormatString=|
      | %<ID>
      | %<Vbase>V
      | %<VLF>pu
      | %<angleLF>deg.
      | %<Name>
  bus59 : powerlib/Measurements/Load Flow Bus  LConnTagsString=a  ID=bus59  Vbase=110000  Vref=1  Vangle=0  VLF=1  angleLF=0
      settings: AttributesFormatString=|
      | %<ID>
      | %<Vbase>V
      | %<VLF>pu
      | %<angleLF>deg.
      | %<Name>
  bus6 : powerlib/Measurements/Load Flow Bus  LConnTagsString=a  ID=bus6  Vbase=110000  Vref=1  Vangle=0  VLF=1  angleLF=0
      settings: AttributesFormatString=|
      | %<ID>
      | %<Vbase>V
      | %<VLF>pu
      | %<angleLF>deg.
      | %<Name>
  bus60 : powerlib/Measurements/Load Flow Bus  LConnTagsString=a  ID=bus60  Vbase=110000  Vref=1  Vangle=0  VLF=1  angleLF=0
      settings: AttributesFormatString=|
      | %<ID>
      | %<Vbase>V
      | %<VLF>pu
      | %<angleLF>deg.
      | %<Name>
  bus61 : powerlib/Measurements/Load Flow Bus  LConnTagsString=a  ID=bus61  Vbase=110000  Vref=1  Vangle=0  VLF=1  angleLF=0
      settings: AttributesFormatString=|
      | %<ID>
      | %<Vbase>V
      | %<VLF>pu
      | %<angleLF>deg.
      | %<Name>
  bus62 : powerlib/Measurements/Load Flow Bus  LConnTagsString=a  ID=bus62  Vbase=110000  Vref=1  Vangle=0  VLF=1  angleLF=0
      settings: AttributesFormatString=|
      | %<ID>
      | %<Vbase>V
      | %<VLF>pu
      | %<angleLF>deg.
      | %<Name>
  bus63 : powerlib/Measurements/Load Flow Bus  LConnTagsString=a  ID=bus63  Vbase=110000  Vref=1  Vangle=0  VLF=1  angleLF=0
      settings: AttributesFormatString=|
      | %<ID>
      | %<Vbase>V
      | %<VLF>pu
      | %<angleLF>deg.
      | %<Name>
  bus64 : powerlib/Measurements/Load Flow Bus  LConnTagsString=a  ID=bus64  Vbase=110000  Vref=1  Vangle=0  VLF=1  angleLF=0
      settings: AttributesFormatString=|
      | %<ID>
      | %<Vbase>V
      | %<VLF>pu
      | %<angleLF>deg.
      | %<Name>
  bus65 : powerlib/Measurements/Load Flow Bus  LConnTagsString=a  ID=bus65  Vbase=110000  Vref=1  Vangle=0  VLF=1  angleLF=0
      settings: AttributesFormatString=|
      | %<ID>
      | %<Vbase>V
      | %<VLF>pu
      | %<angleLF>deg.
      | %<Name>
  bus66 : powerlib/Measurements/Load Flow Bus  LConnTagsString=a  ID=bus66  Vbase=110000  Vref=1  Vangle=0  VLF=1  angleLF=0
      settings: AttributesFormatString=|
      | %<ID>
      | %<Vbase>V
      | %<VLF>pu
      | %<angleLF>deg.
      | %<Name>
  bus67 : powerlib/Measurements/Load Flow Bus  LConnTagsString=a  ID=bus67  Vbase=110000  Vref=1  Vangle=0  VLF=1  angleLF=0
      settings: AttributesFormatString=|
      | %<ID>
      | %<Vbase>V
      | %<VLF>pu
      | %<angleLF>deg.
      | %<Name>
  bus68 : powerlib/Measurements/Load Flow Bus  LConnTagsString=a  ID=bus68  Vbase=110000  Vref=1  Vangle=0  VLF=1  angleLF=0
      settings: AttributesFormatString=|
      | %<ID>
      | %<Vbase>V
      | %<VLF>pu
      | %<angleLF>deg.
      | %<Name>
  bus69 : powerlib/Measurements/Load Flow Bus  LConnTagsString=a  ID=bus69  Vbase=110000  Vref=1  Vangle=0  VLF=1  angleLF=0
      settings: AttributesFormatString=|
      | %<ID>
      | %<Vbase>V
      | %<VLF>pu
      | %<angleLF>deg.
      | %<Name>
  bus7 : powerlib/Measurements/Load Flow Bus  LConnTagsString=a  ID=bus7  Vbase=110000  Vref=1  Vangle=0  VLF=1  angleLF=0
      settings: AttributesFormatString=|
      | %<ID>
      | %<Vbase>V
      | %<VLF>pu
      | %<angleLF>deg.
      | %<Name>
  bus70 : powerlib/Measurements/Load Flow Bus  LConnTagsString=a  ID=bus70  Vbase=110000  Vref=1  Vangle=0  VLF=1  angleLF=0
      settings: AttributesFormatString=|
      | %<ID>
      | %<Vbase>V
      | %<VLF>pu
      | %<angleLF>deg.
      | %<Name>
  bus71 : powerlib/Measurements/Load Flow Bus  LConnTagsString=a  ID=bus71  Vbase=110000  Vref=1  Vangle=0  VLF=1  angleLF=0
      settings: AttributesFormatString=|
      | %<ID>
      | %<Vbase>V
      | %<VLF>pu
      | %<angleLF>deg.
      | %<Name>
  bus72 : powerlib/Measurements/Load Flow Bus  LConnTagsString=a  ID=bus72  Vbase=110000  Vref=1  Vangle=0  VLF=1  angleLF=0
      settings: AttributesFormatString=|
      | %<ID>
      | %<Vbase>V
      | %<VLF>pu
      | %<angleLF>deg.
      | %<Name>
  bus73 : powerlib/Measurements/Load Flow Bus  LConnTagsString=a  ID=bus73  Vbase=110000  Vref=1  Vangle=0  VLF=1  angleLF=0
      settings: AttributesFormatString=|
      | %<ID>
      | %<Vbase>V
      | %<VLF>pu
      | %<angleLF>deg.
      | %<Name>
  bus74 : powerlib/Measurements/Load Flow Bus  LConnTagsString=a  ID=bus74  Vbase=110000  Vref=1  Vangle=0  VLF=1  angleLF=0
      settings: AttributesFormatString=|
      | %<ID>
      | %<Vbase>V
      | %<VLF>pu
      | %<angleLF>deg.
      | %<Name>
  bus75 : powerlib/Measurements/Load Flow Bus  LConnTagsString=a  ID=bus75  Vbase=110000  Vref=1  Vangle=0  VLF=1  angleLF=0
      settings: AttributesFormatString=|
      | %<ID>
      | %<Vbase>V
      | %<VLF>pu
      | %<angleLF>deg.
      | %<Name>
  bus76 : powerlib/Measurements/Load Flow Bus  LConnTagsString=a  ID=bus76  Vbase=110000  Vref=1  Vangle=0  VLF=1  angleLF=0
      settings: AttributesFormatString=|
      | %<ID>
      | %<Vbase>V
      | %<VLF>pu
      | %<angleLF>deg.
      | %<Name>
  bus77 : powerlib/Measurements/Load Flow Bus  LConnTagsString=a  ID=bus77  Vbase=110000  Vref=1  Vangle=0  VLF=1  angleLF=0
      settings: AttributesFormatString=|
      | %<ID>
      | %<Vbase>V
      | %<VLF>pu
      | %<angleLF>deg.
      | %<Name>
  bus78 : powerlib/Measurements/Load Flow Bus  LConnTagsString=a  ID=bus78  Vbase=110000  Vref=1  Vangle=0  VLF=1  angleLF=0
      settings: AttributesFormatString=|
      | %<ID>
      | %<Vbase>V
      | %<VLF>pu
      | %<angleLF>deg.
      | %<Name>
  bus79 : powerlib/Measurements/Load Flow Bus  LConnTagsString=a  ID=bus79  Vbase=110000  Vref=1  Vangle=0  VLF=1  angleLF=0
      settings: AttributesFormatString=|
      | %<ID>
      | %<Vbase>V
      | %<VLF>pu
      | %<angleLF>deg.
      | %<Name>
  bus8 : powerlib/Measurements/Load Flow Bus  LConnTagsString=a  ID=bus8  Vbase=110000  Vref=1  Vangle=0  VLF=1  angleLF=0
      settings: AttributesFormatString=|
      | %<ID>
      | %<Vbase>V
      | %<VLF>pu
      | %<angleLF>deg.
      | %<Name>
  bus80 : powerlib/Measurements/Load Flow Bus  LConnTagsString=a  ID=bus80  Vbase=110000  Vref=1  Vangle=0  VLF=1  angleLF=0
      settings: AttributesFormatString=|
      | %<ID>
      | %<Vbase>V
      | %<VLF>pu
      | %<angleLF>deg.
      | %<Name>
  bus81 : powerlib/Measurements/Load Flow Bus  LConnTagsString=a  ID=bus81  Vbase=110000  Vref=1  Vangle=0  VLF=1  angleLF=0
      settings: AttributesFormatString=|
      | %<ID>
      | %<Vbase>V
      | %<VLF>pu
      | %<angleLF>deg.
      | %<Name>
  bus82 : powerlib/Measurements/Load Flow Bus  LConnTagsString=a  ID=bus82  Vbase=110000  Vref=1  Vangle=0  VLF=1  angleLF=0
      settings: AttributesFormatString=|
      | %<ID>
      | %<Vbase>V
      | %<VLF>pu
      | %<angleLF>deg.
      | %<Name>
  bus83 : powerlib/Measurements/Load Flow Bus  LConnTagsString=a  ID=bus83  Vbase=110000  Vref=1  Vangle=0  VLF=1  angleLF=0
      settings: AttributesFormatString=|
      | %<ID>
      | %<Vbase>V
      | %<VLF>pu
      | %<angleLF>deg.
      | %<Name>
  bus84 : powerlib/Measurements/Load Flow Bus  LConnTagsString=a  ID=bus84  Vbase=110000  Vref=1  Vangle=0  VLF=1  angleLF=0
      settings: AttributesFormatString=|
      | %<ID>
      | %<Vbase>V
      | %<VLF>pu
      | %<angleLF>deg.
      | %<Name>
  bus85 : powerlib/Measurements/Load Flow Bus  LConnTagsString=a  ID=bus85  Vbase=110000  Vref=1  Vangle=0  VLF=1  angleLF=0
      settings: AttributesFormatString=|
      | %<ID>
      | %<Vbase>V
      | %<VLF>pu
      | %<angleLF>deg.
      | %<Name>
  bus86 : powerlib/Measurements/Load Flow Bus  LConnTagsString=a  ID=bus86  Vbase=110000  Vref=1  Vangle=0  VLF=1  angleLF=0
      settings: AttributesFormatString=|
      | %<ID>
      | %<Vbase>V
      | %<VLF>pu
      | %<angleLF>deg.
      | %<Name>
  bus87 : powerlib/Measurements/Load Flow Bus  LConnTagsString=a  ID=bus87  Vbase=110000  Vref=1  Vangle=0  VLF=1  angleLF=0
      settings: AttributesFormatString=|
      | %<ID>
      | %<Vbase>V
      | %<VLF>pu
      | %<angleLF>deg.
      | %<Name>
  bus88 : powerlib/Measurements/Load Flow Bus  LConnTagsString=a  ID=bus88  Vbase=110000  Vref=1  Vangle=0  VLF=1  angleLF=0
      settings: AttributesFormatString=|
      | %<ID>
      | %<Vbase>V
      | %<VLF>pu
      | %<angleLF>deg.
      | %<Name>
  bus89 : powerlib/Measurements/Load Flow Bus  LConnTagsString=a  ID=bus89  Vbase=110000  Vref=1  Vangle=0  VLF=1  angleLF=0
      settings: AttributesFormatString=|
      | %<ID>
      | %<Vbase>V
      | %<VLF>pu
      | %<angleLF>deg.
      | %<Name>
  bus9 : powerlib/Measurements/Load Flow Bus  LConnTagsString=a  ID=bus9  Vbase=110000  Vref=1  Vangle=0  VLF=1  angleLF=0
      settings: AttributesFormatString=|
      | %<ID>
      | %<Vbase>V
      | %<VLF>pu
      | %<angleLF>deg.
      | %<Name>
  bus90 : powerlib/Measurements/Load Flow Bus  LConnTagsString=a  ID=bus90  Vbase=110000  Vref=1  Vangle=0  VLF=1  angleLF=0
      settings: AttributesFormatString=|
      | %<ID>
      | %<Vbase>V
      | %<VLF>pu
      | %<angleLF>deg.
      | %<Name>
  bus91 : powerlib/Measurements/Load Flow Bus  LConnTagsString=a  ID=bus91  Vbase=110000  Vref=1  Vangle=0  VLF=1  angleLF=0
      settings: AttributesFormatString=|
      | %<ID>
      | %<Vbase>V
      | %<VLF>pu
      | %<angleLF>deg.
      | %<Name>
  bus92 : powerlib/Measurements/Load Flow Bus  LConnTagsString=a  ID=bus92  Vbase=110000  Vref=1  Vangle=0  VLF=1  angleLF=0
      settings: AttributesFormatString=|
      | %<ID>
      | %<Vbase>V
      | %<VLF>pu
      | %<angleLF>deg.
      | %<Name>
  bus93 : powerlib/Measurements/Load Flow Bus  LConnTagsString=a  ID=bus93  Vbase=110000  Vref=1  Vangle=0  VLF=1  angleLF=0
      settings: AttributesFormatString=|
      | %<ID>
      | %<Vbase>V
      | %<VLF>pu
      | %<angleLF>deg.
      | %<Name>
  bus94 : powerlib/Measurements/Load Flow Bus  LConnTagsString=a  ID=bus94  Vbase=110000  Vref=1  Vangle=0  VLF=1  angleLF=0
      settings: AttributesFormatString=|
      | %<ID>
      | %<Vbase>V
      | %<VLF>pu
      | %<angleLF>deg.
      | %<Name>
  bus95 : powerlib/Measurements/Load Flow Bus  LConnTagsString=a  ID=bus95  Vbase=110000  Vref=1  Vangle=0  VLF=1  angleLF=0
      settings: AttributesFormatString=|
      | %<ID>
      | %<Vbase>V
      | %<VLF>pu
      | %<angleLF>deg.
      | %<Name>
  bus96 : powerlib/Measurements/Load Flow Bus  LConnTagsString=a  ID=bus96  Vbase=110000  Vref=1  Vangle=0  VLF=1  angleLF=0
      settings: AttributesFormatString=|
      | %<ID>
      | %<Vbase>V
      | %<VLF>pu
      | %<angleLF>deg.
      | %<Name>
  bus97 : powerlib/Measurements/Load Flow Bus  LConnTagsString=a  ID=bus97  Vbase=110000  Vref=1  Vangle=0  VLF=1  angleLF=0
      settings: AttributesFormatString=|
      | %<ID>
      | %<Vbase>V
      | %<VLF>pu
      | %<angleLF>deg.
      | %<Name>
  bus98 : powerlib/Measurements/Load Flow Bus  LConnTagsString=a  ID=bus98  Vbase=110000  Vref=1  Vangle=0  VLF=1  angleLF=0
      settings: AttributesFormatString=|
      | %<ID>
      | %<Vbase>V
      | %<VLF>pu
      | %<angleLF>deg.
      | %<Name>
  bus99 : powerlib/Measurements/Load Flow Bus  LConnTagsString=a  ID=bus99  Vbase=110000  Vref=1  Vangle=0  VLF=1  angleLF=0
      settings: AttributesFormatString=|
      | %<ID>
      | %<Vbase>V
      | %<VLF>pu
      | %<angleLF>deg.
      | %<Name>
  powergui : powerlib/powergui  Priority=1  SimulationMode=Continuous  SolverType=Tustin  SampleTime=50e-6  frequency=60  SPID=off  DisableSnubberDevices=off  DisableRonSwitches=off  DisableVfSwitches=off  SwTol=0  Interpol=off  DisplayEquations=off  Ts=0  methode=off  frequencyindice=60  Pbase=100e6  ErrMax=1e-4  Iterations=50  UnitsV=kV  UnitsW=MW  FunctionMessages=off  echomessages=off  HookPort=off  EnableUseOfTLC=off  x0status=blocks  RestoreLinks=warning  ResistiveCurrentMeasurement=off  Frange=[0:2:500]  Ylog=off  Xlog=on  ShowGrid=off  save=off  variable=ZData  structure=0  ZoomFFT=off  StartTime=0.0  cycles=1  DisplayStyle=1  fundamental=60  FreqAxis=off  MaxFrequency=1000  frequencyindicesteady=1  RmsSteady=1  display=off
  connections:
  _CN_172590080_110000_CN_172178556_110000/LConn1 -- T_172590080__/LConn1 -- _CN_172590080_110000_CN_172394941_110000/LConn1 -- _CN_172590080_110000_CN_214227031_110000/LConn1 -- _CN_172590080_110000_CN_158244489_110000/LConn1 -- _CN_172590080_110000_CN_172590115_110000/LConn1 -- _CN_172590080_110000_CN_172394923_110000/LConn1 -- _CN_172590080_110000_CN_172590081_110000/LConn1 -- _CN_172590080_110000_CN_172590100_110000/LConn1 -- _CN_172590080_110000_CN_172590098_110000/LConn1 -- _CN_172590080_110000_CN_135895688_110000/LConn1 -- _CN_172590080_110000_CN_172590101_110000/LConn1 -- _CN_172590080_110000_CN_172590105_110000/LConn1 -- _CN_172590080_110000_CN_257169562_110000/LConn1 -- _CN_172590080_110000_CN_173765447_110000/LConn1 -- _CN_172590080_110000_CN_172590075_110000/LConn1 -- _CN_172590080_110000_CN_172590076_110000/LConn1 -- _CN_172590080_110000_CN_172590116_110000/LConn1 -- _CN_172590080_110000_CN_172445101_110000/LConn1 -- _CN_172590080_110000_CN_172590051_110000/LConn1 -- _CN_172590080_110000_CN_172590088_110000/LConn1 -- _CN_172590080_110000_CN_265807988_110000/LConn1 -- _CN_172590080_110000_CN_215671382_110000/LConn1 -- _CN_172590080_110000_CN_172445107_110000/LConn1 -- _CN_172590080_110000_CN_172445089_110000/LConn1 -- _CN_172590080_110000_CN_172445103_110000/LConn1 -- _CN_172590080_110000_CN_172019127_110000/LConn1
  _CN_172590080_110000_CN_172178556_110000/LConn2 -- T_172590080__/LConn2 -- _CN_172590080_110000_CN_172394941_110000/LConn2 -- _CN_172590080_110000_CN_214227031_110000/LConn2 -- _CN_172590080_110000_CN_158244489_110000/LConn2 -- _CN_172590080_110000_CN_172590115_110000/LConn2 -- _CN_172590080_110000_CN_172394923_110000/LConn2 -- _CN_172590080_110000_CN_172590081_110000/LConn2 -- _CN_172590080_110000_CN_172590100_110000/LConn2 -- _CN_172590080_110000_CN_172590098_110000/LConn2 -- _CN_172590080_110000_CN_135895688_110000/LConn2 -- _CN_172590080_110000_CN_172590101_110000/LConn2 -- _CN_172590080_110000_CN_172590105_110000/LConn2 -- _CN_172590080_110000_CN_257169562_110000/LConn2 -- _CN_172590080_110000_CN_173765447_110000/LConn2 -- _CN_172590080_110000_CN_172590075_110000/LConn2 -- _CN_172590080_110000_CN_172590076_110000/LConn2 -- _CN_172590080_110000_CN_172590116_110000/LConn2 -- _CN_172590080_110000_CN_172445101_110000/LConn2 -- _CN_172590080_110000_CN_172590051_110000/LConn2 -- _CN_172590080_110000_CN_172590088_110000/LConn2 -- _CN_172590080_110000_CN_265807988_110000/LConn2 -- _CN_172590080_110000_CN_215671382_110000/LConn2 -- _CN_172590080_110000_CN_172445107_110000/LConn2 -- _CN_172590080_110000_CN_172445089_110000/LConn2 -- _CN_172590080_110000_CN_172445103_110000/LConn2 -- _CN_172590080_110000_CN_172019127_110000/LConn2
  _CN_172590080_110000_CN_172178556_110000/LConn3 -- T_172590080__/LConn3 -- _CN_172590080_110000_CN_172394941_110000/LConn3 -- _CN_172590080_110000_CN_214227031_110000/LConn3 -- _CN_172590080_110000_CN_158244489_110000/LConn3 -- _CN_172590080_110000_CN_172590115_110000/LConn3 -- _CN_172590080_110000_CN_172394923_110000/LConn3 -- _CN_172590080_110000_CN_172590081_110000/LConn3 -- bus1/LConn1 -- _CN_172590080_110000_CN_172590100_110000/LConn3 -- _CN_172590080_110000_CN_172590098_110000/LConn3 -- _CN_172590080_110000_CN_135895688_110000/LConn3 -- _CN_172590080_110000_CN_172590101_110000/LConn3 -- _CN_172590080_110000_CN_172590105_110000/LConn3 -- _CN_172590080_110000_CN_257169562_110000/LConn3 -- _CN_172590080_110000_CN_173765447_110000/LConn3 -- _CN_172590080_110000_CN_172590075_110000/LConn3 -- _CN_172590080_110000_CN_172590076_110000/LConn3 -- _CN_172590080_110000_CN_172590116_110000/LConn3 -- _CN_172590080_110000_CN_172445101_110000/LConn3 -- _CN_172590080_110000_CN_172590051_110000/LConn3 -- _CN_172590080_110000_CN_172590088_110000/LConn3 -- _CN_172590080_110000_CN_265807988_110000/LConn3 -- _CN_172590080_110000_CN_215671382_110000/LConn3 -- _CN_172590080_110000_CN_172445107_110000/LConn3 -- _CN_172590080_110000_CN_172445089_110000/LConn3 -- _CN_172590080_110000_CN_172445103_110000/LConn3 -- _CN_172590080_110000_CN_172019127_110000/LConn3
  _CN_172590080_110000_CN_172178556_110000/RConn1 -- T_172178556__/LConn1 -- _CN_172178556_110000_CN_166814917_110000/LConn1
  _CN_172590080_110000_CN_172178556_110000/RConn2 -- T_172178556__/LConn2 -- _CN_172178556_110000_CN_166814917_110000/LConn2
  _CN_172590080_110000_CN_172178556_110000/RConn3 -- T_172178556__/LConn3 -- _CN_172178556_110000_CN_166814917_110000/LConn3 -- bus2/LConn1
  _CN_172590080_110000_CN_172590100_110000/RConn1 -- T_172590100__Rokų_TP/LConn1 -- _CN_172590100_110000_CN_173612890_110000/LConn1
  _CN_172590080_110000_CN_172590100_110000/RConn2 -- T_172590100__Rokų_TP/LConn2 -- _CN_172590100_110000_CN_173612890_110000/LConn2
  _CN_172590080_110000_CN_172590100_110000/RConn3 -- T_172590100__Rokų_TP/LConn3 -- _CN_172590100_110000_CN_173612890_110000/LConn3 -- bus3/LConn1
  T_172590098__Drobės_TP/LConn1 -- _CN_172590080_110000_CN_172590098_110000/RConn1
  T_172590098__Drobės_TP/LConn2 -- _CN_172590080_110000_CN_172590098_110000/RConn2
  _CN_172590080_110000_CN_172590098_110000/RConn3 -- T_172590098__Drobės_TP/LConn3 -- bus4/LConn1
  T_135895688__Palemono_Traukos_TP/LConn1 -- _CN_172590080_110000_CN_135895688_110000/RConn1
  T_135895688__Palemono_Traukos_TP/LConn2 -- _CN_172590080_110000_CN_135895688_110000/RConn2
  _CN_172590080_110000_CN_135895688_110000/RConn3 -- T_135895688__Palemono_Traukos_TP/LConn3 -- bus5/LConn1
  T_172590101__Petrašiūnų_TP/LConn1 -- _CN_172590080_110000_CN_172590101_110000/RConn1
  T_172590101__Petrašiūnų_TP/LConn2 -- _CN_172590080_110000_CN_172590101_110000/RConn2
  _CN_172590080_110000_CN_172590101_110000/RConn3 -- T_172590101__Petrašiūnų_TP/LConn3 -- bus6/LConn1
  T_172590105__Ketaus_TP/LConn1 -- _CN_172590080_110000_CN_172590105_110000/RConn1
  T_172590105__Ketaus_TP/LConn2 -- _CN_172590080_110000_CN_172590105_110000/RConn2
  _CN_172590080_110000_CN_172590105_110000/RConn3 -- T_172590105__Ketaus_TP/LConn3 -- bus7/LConn1
  _CN_172590080_110000_CN_257169562_110000/RConn1 -- T_257169562__Kauno_transformatorinė_pastotė/RConn1 -- _CN_88726161_110000_CN_257169562_110000/LConn1 -- _CN_171868832_110000_CN_257169562_110000/LConn1 -- L_257169562/LConn1
  _CN_172590080_110000_CN_257169562_110000/RConn2 -- T_257169562__Kauno_transformatorinė_pastotė/RConn2 -- _CN_88726161_110000_CN_257169562_110000/LConn2 -- _CN_171868832_110000_CN_257169562_110000/LConn2 -- L_257169562/LConn2
  _CN_172590080_110000_CN_257169562_110000/RConn3 -- T_257169562__Kauno_transformatorinė_pastotė/RConn3 -- _CN_88726161_110000_CN_257169562_110000/LConn3 -- _CN_171868832_110000_CN_257169562_110000/LConn3 -- L_257169562/LConn3 -- bus8/LConn1
  T_173765447__Pluošto_TP/LConn1 -- _CN_172590080_110000_CN_173765447_110000/RConn1
  T_173765447__Pluošto_TP/LConn2 -- _CN_172590080_110000_CN_173765447_110000/RConn2
  _CN_172590080_110000_CN_173765447_110000/RConn3 -- T_173765447__Pluošto_TP/LConn3 -- bus9/LConn1
  T_172590075__Žasmos_TP/LConn1 -- _CN_172590080_110000_CN_172590075_110000/RConn1
  T_172590075__Žasmos_TP/LConn2 -- _CN_172590080_110000_CN_172590075_110000/RConn2
  _CN_172590080_110000_CN_172590075_110000/RConn3 -- T_172590075__Žasmos_TP/LConn3 -- bus10/LConn1
  T_172590076__/LConn1 -- _CN_172590080_110000_CN_172590076_110000/RConn1
  T_172590076__/LConn2 -- _CN_172590080_110000_CN_172590076_110000/RConn2
  _CN_172590080_110000_CN_172590076_110000/RConn3 -- T_172590076__/LConn3 -- bus11/LConn1
  T_172590116__/LConn1 -- _CN_172590080_110000_CN_172590116_110000/RConn1
  T_172590116__/LConn2 -- _CN_172590080_110000_CN_172590116_110000/RConn2
  _CN_172590080_110000_CN_172590116_110000/RConn3 -- T_172590116__/LConn3 -- bus12/LConn1
  T_172445101__/LConn1 -- _CN_172590080_110000_CN_172445101_110000/RConn1
  T_172445101__/LConn2 -- _CN_172590080_110000_CN_172445101_110000/RConn2
  _CN_172590080_110000_CN_172445101_110000/RConn3 -- T_172445101__/LConn3 -- bus13/LConn1
  _CN_172590080_110000_CN_172590051_110000/RConn1 -- T_172590051__/RConn1 -- _CN_172445089_110000_CN_172590051_110000/LConn1 -- L_172590051/LConn1 -- _CN_172590096_110000_CN_172590051_110000/LConn1 -- _CN_172590097_110000_CN_172590051_110000/LConn1 -- _CN_172178550_110000_CN_172590051_110000/LConn1
  _CN_172590080_110000_CN_172590051_110000/RConn2 -- T_172590051__/RConn2 -- _CN_172445089_110000_CN_172590051_110000/LConn2 -- L_172590051/LConn2 -- _CN_172590096_110000_CN_172590051_110000/LConn2 -- _CN_172590097_110000_CN_172590051_110000/LConn2 -- _CN_172178550_110000_CN_172590051_110000/LConn2
  _CN_172590080_110000_CN_172590051_110000/RConn3 -- T_172590051__/RConn3 -- _CN_172445089_110000_CN_172590051_110000/LConn3 -- L_172590051/LConn3 -- bus14/LConn1 -- _CN_172590096_110000_CN_172590051_110000/LConn3 -- _CN_172590097_110000_CN_172590051_110000/LConn3 -- _CN_172178550_110000_CN_172590051_110000/LConn3
  T_172590088__/LConn1 -- _CN_172590080_110000_CN_172590088_110000/RConn1
  T_172590088__/LConn2 -- _CN_172590080_110000_CN_172590088_110000/RConn2
  _CN_172590080_110000_CN_172590088_110000/RConn3 -- T_172590088__/LConn3 -- bus15/LConn1
  T_265807988__/LConn1 -- _CN_172590080_110000_CN_265807988_110000/RConn1
  T_265807988__/LConn2 -- _CN_172590080_110000_CN_265807988_110000/RConn2
  _CN_172590080_110000_CN_265807988_110000/RConn3 -- T_265807988__/LConn3 -- bus16/LConn1
  _CN_172590080_110000_CN_215671382_110000/RConn1 -- T_215671382__/LConn1 -- _CN_215671382_110000_CN_172019117_110000/LConn1 -- _CN_215671382_110000_CN_172019087_110000/LConn1
  _CN_172590080_110000_CN_215671382_110000/RConn2 -- T_215671382__/LConn2 -- _CN_215671382_110000_CN_172019117_110000/LConn2 -- _CN_215671382_110000_CN_172019087_110000/LConn2
  _CN_172590080_110000_CN_215671382_110000/RConn3 -- T_215671382__/LConn3 -- _CN_215671382_110000_CN_172019117_110000/LConn3 -- _CN_215671382_110000_CN_172019087_110000/LConn3 -- bus17/LConn1
  T_172445107__/LConn1 -- _CN_172590080_110000_CN_172445107_110000/RConn1
  T_172445107__/LConn2 -- _CN_172590080_110000_CN_172445107_110000/RConn2
  _CN_172590080_110000_CN_172445107_110000/RConn3 -- T_172445107__/LConn3 -- bus18/LConn1
  _CN_172590080_110000_CN_172445089_110000/RConn1 -- T_172445089__/LConn1 -- _CN_172445089_110000_CN_172590051_110000/RConn1 -- _CN_172445089_110000_CN_172445102_110000/LConn1
  _CN_172590080_110000_CN_172445089_110000/RConn2 -- T_172445089__/LConn2 -- _CN_172445089_110000_CN_172590051_110000/RConn2 -- _CN_172445089_110000_CN_172445102_110000/LConn2
  _CN_172590080_110000_CN_172445089_110000/RConn3 -- T_172445089__/LConn3 -- _CN_172445089_110000_CN_172590051_110000/RConn3 -- bus19/LConn1 -- _CN_172445089_110000_CN_172445102_110000/LConn3
  T_172445103__/LConn1 -- _CN_172590080_110000_CN_172445103_110000/RConn1
  T_172445103__/LConn2 -- _CN_172590080_110000_CN_172445103_110000/RConn2
  _CN_172590080_110000_CN_172445103_110000/RConn3 -- T_172445103__/LConn3 -- bus20/LConn1
  T_172019127__/LConn1 -- _CN_172590080_110000_CN_172019127_110000/RConn1
  T_172019127__/LConn2 -- _CN_172590080_110000_CN_172019127_110000/RConn2
  _CN_172590080_110000_CN_172019127_110000/RConn3 -- T_172019127__/LConn3 -- bus21/LConn1
  _CN_172590080_110000_CN_172394941_110000/RConn1 -- T_172394941__/LConn1 -- _CN_221105370_110000_CN_172394941_110000/LConn1
  _CN_172590080_110000_CN_172394941_110000/RConn2 -- T_172394941__/LConn2 -- _CN_221105370_110000_CN_172394941_110000/LConn2
  _CN_172590080_110000_CN_172394941_110000/RConn3 -- T_172394941__/LConn3 -- _CN_221105370_110000_CN_172394941_110000/LConn3 -- bus22/LConn1
  T_214227031__/LConn1 -- _CN_172590080_110000_CN_214227031_110000/RConn1
  T_214227031__/LConn2 -- _CN_172590080_110000_CN_214227031_110000/RConn2
  _CN_172590080_110000_CN_214227031_110000/RConn3 -- T_214227031__/LConn3 -- bus23/LConn1
  T_158244489__Palemono_TP/LConn1 -- _CN_172590080_110000_CN_158244489_110000/RConn1
  T_158244489__Palemono_TP/LConn2 -- _CN_172590080_110000_CN_158244489_110000/RConn2
  _CN_172590080_110000_CN_158244489_110000/RConn3 -- T_158244489__Palemono_TP/LConn3 -- bus24/LConn1
  _CN_172590080_110000_CN_172590115_110000/RConn1 -- T_172590115_330000;110000;fixme_/RConn1 -- L_172590115/LConn1
  _CN_172590080_110000_CN_172590115_110000/RConn2 -- T_172590115_330000;110000;fixme_/RConn2 -- L_172590115/LConn2
  _CN_172590080_110000_CN_172590115_110000/RConn3 -- T_172590115_330000;110000;fixme_/RConn3 -- L_172590115/LConn3 -- bus25/LConn1
  T_172394923__/LConn1 -- _CN_172590080_110000_CN_172394923_110000/RConn1
  T_172394923__/LConn2 -- _CN_172590080_110000_CN_172394923_110000/RConn2
  _CN_172590080_110000_CN_172394923_110000/RConn3 -- T_172394923__/LConn3 -- bus26/LConn1
  T_172590081__/LConn1 -- _CN_172590080_110000_CN_172590081_110000/RConn1
  T_172590081__/LConn2 -- _CN_172590080_110000_CN_172590081_110000/RConn2
  _CN_172590080_110000_CN_172590081_110000/RConn3 -- T_172590081__/LConn3 -- bus27/LConn1
  _CN_258321412_110000_CN_214649882_110000/LConn1 -- T_258321412__/RConn1 -- _CN_258321412_110000_CN_172019085_110000/LConn1 -- _CN_258321412_110000_CN_174586802_110000/LConn1 -- _CN_258321412_110000_CN_172019051_110000/LConn1 -- _CN_258321412_110000_CN_214649879_110000/LConn1 -- _CN_258321412_110000_CN_171809316_110000/LConn1 -- L_258321412/LConn1 -- _CN_258321412_110000_CN_194082693_110000/LConn1 -- _CN_258321412_110000_CN_212007661_110000/LConn1 -- _CN_258321412_110000_CN_214674623_110000/LConn1 -- _CN_258321412_110000_CN_172019090_110000/LConn1 -- _CN_258321412_110000_CN_210995832_110000/LConn1
  _CN_258321412_110000_CN_214649882_110000/LConn2 -- T_258321412__/RConn2 -- _CN_258321412_110000_CN_172019085_110000/LConn2 -- _CN_258321412_110000_CN_174586802_110000/LConn2 -- _CN_258321412_110000_CN_172019051_110000/LConn2 -- _CN_258321412_110000_CN_214649879_110000/LConn2 -- _CN_258321412_110000_CN_171809316_110000/LConn2 -- L_258321412/LConn2 -- _CN_258321412_110000_CN_194082693_110000/LConn2 -- _CN_258321412_110000_CN_212007661_110000/LConn2 -- _CN_258321412_110000_CN_214674623_110000/LConn2 -- _CN_258321412_110000_CN_172019090_110000/LConn2 -- _CN_258321412_110000_CN_210995832_110000/LConn2
  _CN_258321412_110000_CN_214649882_110000/LConn3 -- T_258321412__/RConn3 -- _CN_258321412_110000_CN_172019085_110000/LConn3 -- _CN_258321412_110000_CN_174586802_110000/LConn3 -- _CN_258321412_110000_CN_172019051_110000/LConn3 -- _CN_258321412_110000_CN_214649879_110000/LConn3 -- _CN_258321412_110000_CN_171809316_110000/LConn3 -- L_258321412/LConn3 -- bus28/LConn1 -- _CN_258321412_110000_CN_194082693_110000/LConn3 -- _CN_258321412_110000_CN_212007661_110000/LConn3 -- _CN_258321412_110000_CN_214674623_110000/LConn3 -- _CN_258321412_110000_CN_172019090_110000/LConn3 -- _CN_258321412_110000_CN_210995832_110000/LConn3
  T_214649882__/LConn1 -- _CN_258321412_110000_CN_214649882_110000/RConn1
  T_214649882__/LConn2 -- _CN_258321412_110000_CN_214649882_110000/RConn2
  _CN_258321412_110000_CN_214649882_110000/RConn3 -- T_214649882__/LConn3 -- bus29/LConn1
  _CN_258321412_110000_CN_172019090_110000/RConn1 -- T_172019090__/LConn1 -- _CN_172018985_110000_CN_172019090_110000/LConn1
  _CN_258321412_110000_CN_172019090_110000/RConn2 -- T_172019090__/LConn2 -- _CN_172018985_110000_CN_172019090_110000/LConn2
  _CN_258321412_110000_CN_172019090_110000/RConn3 -- T_172019090__/LConn3 -- _CN_172018985_110000_CN_172019090_110000/LConn3 -- bus30/LConn1
  T_210995832__/LConn1 -- _CN_258321412_110000_CN_210995832_110000/RConn1
  T_210995832__/LConn2 -- _CN_258321412_110000_CN_210995832_110000/RConn2
  _CN_258321412_110000_CN_210995832_110000/RConn3 -- T_210995832__/LConn3 -- bus31/LConn1
  _CN_258321412_110000_CN_194082693_110000/RConn1 -- T_194082693__/LConn1 -- _CN_239589747_110000_CN_194082693_110000/LConn1
  _CN_258321412_110000_CN_194082693_110000/RConn2 -- T_194082693__/LConn2 -- _CN_239589747_110000_CN_194082693_110000/LConn2
  _CN_258321412_110000_CN_194082693_110000/RConn3 -- T_194082693__/LConn3 -- _CN_239589747_110000_CN_194082693_110000/LConn3 -- bus32/LConn1
  T_212007661_110000;fixme_/LConn1 -- _CN_258321412_110000_CN_212007661_110000/RConn1
  T_212007661_110000;fixme_/LConn2 -- _CN_258321412_110000_CN_212007661_110000/RConn2
  _CN_258321412_110000_CN_212007661_110000/RConn3 -- T_212007661_110000;fixme_/LConn3 -- bus33/LConn1
  T_214674623__/LConn1 -- _CN_258321412_110000_CN_214674623_110000/RConn1
  T_214674623__/LConn2 -- _CN_258321412_110000_CN_214674623_110000/RConn2
  _CN_258321412_110000_CN_214674623_110000/RConn3 -- T_214674623__/LConn3 -- bus34/LConn1
  T_172019085__/LConn1 -- _CN_258321412_110000_CN_172019085_110000/RConn1
  T_172019085__/LConn2 -- _CN_258321412_110000_CN_172019085_110000/RConn2
  _CN_258321412_110000_CN_172019085_110000/RConn3 -- T_172019085__/LConn3 -- bus35/LConn1
  T_174586802__/LConn1 -- _CN_258321412_110000_CN_174586802_110000/RConn1
  T_174586802__/LConn2 -- _CN_258321412_110000_CN_174586802_110000/RConn2
  _CN_258321412_110000_CN_174586802_110000/RConn3 -- T_174586802__/LConn3 -- bus36/LConn1
  T_172019051__/LConn1 -- _CN_258321412_110000_CN_172019051_110000/RConn1
  T_172019051__/LConn2 -- _CN_258321412_110000_CN_172019051_110000/RConn2
  _CN_258321412_110000_CN_172019051_110000/RConn3 -- T_172019051__/LConn3 -- bus37/LConn1
  T_214649879__/LConn1 -- _CN_258321412_110000_CN_214649879_110000/RConn1
  T_214649879__/LConn2 -- _CN_258321412_110000_CN_214649879_110000/RConn2
  _CN_258321412_110000_CN_214649879_110000/RConn3 -- T_214649879__/LConn3 -- bus38/LConn1
  _CN_258321412_110000_CN_171809316_110000/RConn1 -- T_171809316__/LConn1 -- _CN_214455329_110000_CN_171809316_110000/LConn1
  _CN_258321412_110000_CN_171809316_110000/RConn2 -- T_171809316__/LConn2 -- _CN_214455329_110000_CN_171809316_110000/LConn2
  _CN_258321412_110000_CN_171809316_110000/RConn3 -- T_171809316__/LConn3 -- _CN_214455329_110000_CN_171809316_110000/LConn3 -- bus39/LConn1
  _CN_103275527_110000_CN_103275559_110000/LConn1 -- T_103275527__/LConn1 -- _CN_103275527_110000_CN_103275551_110000/LConn1 -- _CN_103275527_110000_CN_209204254_110000/LConn1 -- _CN_103275527_110000_CN_103560163_110000/LConn1 -- _CN_103275527_110000_CN_124462106_110000/LConn1 -- _CN_103275527_110000_CN_171630121_110000/LConn1
  _CN_103275527_110000_CN_103275559_110000/LConn2 -- T_103275527__/LConn2 -- _CN_103275527_110000_CN_103275551_110000/LConn2 -- _CN_103275527_110000_CN_209204254_110000/LConn2 -- _CN_103275527_110000_CN_103560163_110000/LConn2 -- _CN_103275527_110000_CN_124462106_110000/LConn2 -- _CN_103275527_110000_CN_171630121_110000/LConn2
  _CN_103275527_110000_CN_103275559_110000/LConn3 -- T_103275527__/LConn3 -- _CN_103275527_110000_CN_103275551_110000/LConn3 -- _CN_103275527_110000_CN_209204254_110000/LConn3 -- _CN_103275527_110000_CN_103560163_110000/LConn3 -- _CN_103275527_110000_CN_124462106_110000/LConn3 -- _CN_103275527_110000_CN_171630121_110000/LConn3 -- bus40/LConn1
  _CN_103275527_110000_CN_103275559_110000/RConn1 -- T_103275559__/LConn1 -- _CN_103275559_110000_CN_103275575_110000/LConn1
  _CN_103275527_110000_CN_103275559_110000/RConn2 -- T_103275559__/LConn2 -- _CN_103275559_110000_CN_103275575_110000/LConn2
  _CN_103275527_110000_CN_103275559_110000/RConn3 -- T_103275559__/LConn3 -- _CN_103275559_110000_CN_103275575_110000/LConn3 -- bus41/LConn1
  T_103275551__/LConn1 -- _CN_103275527_110000_CN_103275551_110000/RConn1
  T_103275551__/LConn2 -- _CN_103275527_110000_CN_103275551_110000/RConn2
  _CN_103275527_110000_CN_103275551_110000/RConn3 -- T_103275551__/LConn3 -- bus42/LConn1
  T_209204254__/LConn1 -- _CN_103275527_110000_CN_209204254_110000/RConn1
  T_209204254__/LConn2 -- _CN_103275527_110000_CN_209204254_110000/RConn2
  _CN_103275527_110000_CN_209204254_110000/RConn3 -- T_209204254__/LConn3 -- bus43/LConn1
  _CN_103275527_110000_CN_103560163_110000/RConn1 -- T_103560163__/LConn1 -- _CN_171630144_110000_CN_103560163_110000/LConn1
  _CN_103275527_110000_CN_103560163_110000/RConn2 -- T_103560163__/LConn2 -- _CN_171630144_110000_CN_103560163_110000/LConn2
  _CN_103275527_110000_CN_103560163_110000/RConn3 -- T_103560163__/LConn3 -- _CN_171630144_110000_CN_103560163_110000/LConn3 -- bus44/LConn1
  T_124462106__/LConn1 -- _CN_103275527_110000_CN_124462106_110000/RConn1
  T_124462106__/LConn2 -- _CN_103275527_110000_CN_124462106_110000/RConn2
  _CN_103275527_110000_CN_124462106_110000/RConn3 -- T_124462106__/LConn3 -- bus45/LConn1
  _CN_103275527_110000_CN_171630121_110000/RConn1 -- T_171630121__/LConn1 -- _CN_171630121_110000_CN_207755730_110000/LConn1 -- _CN_171630121_110000_CN_207755729_110000/LConn1 -- _CN_171630121_110000_CN_103554499_110000/LConn1
  _CN_103275527_110000_CN_171630121_110000/RConn2 -- T_171630121__/LConn2 -- _CN_171630121_110000_CN_207755730_110000/LConn2 -- _CN_171630121_110000_CN_207755729_110000/LConn2 -- _CN_171630121_110000_CN_103554499_110000/LConn2
  _CN_103275527_110000_CN_171630121_110000/RConn3 -- T_171630121__/LConn3 -- _CN_171630121_110000_CN_207755730_110000/LConn3 -- _CN_171630121_110000_CN_207755729_110000/LConn3 -- bus46/LConn1 -- _CN_171630121_110000_CN_103554499_110000/LConn3
  _CN_142782984_110000_CN_173582225_110000/LConn1 -- T_142782984__/LConn1 -- _CN_142782984_110000_CN_153249112_110000/LConn1 -- _CN_142782984_110000_CN_25698690_110000/LConn1
  _CN_142782984_110000_CN_173582225_110000/LConn2 -- T_142782984__/LConn2 -- _CN_142782984_110000_CN_153249112_110000/LConn2 -- _CN_142782984_110000_CN_25698690_110000/LConn2
  _CN_142782984_110000_CN_173582225_110000/LConn3 -- T_142782984__/LConn3 -- _CN_142782984_110000_CN_153249112_110000/LConn3 -- _CN_142782984_110000_CN_25698690_110000/LConn3 -- bus47/LConn1
  _CN_142782984_110000_CN_173582225_110000/RConn1 -- T_173582225__/LConn1 -- _CN_220915873_110000_CN_173582225_110000/LConn1
  _CN_142782984_110000_CN_173582225_110000/RConn2 -- T_173582225__/LConn2 -- _CN_220915873_110000_CN_173582225_110000/LConn2
  _CN_142782984_110000_CN_173582225_110000/RConn3 -- T_173582225__/LConn3 -- _CN_220915873_110000_CN_173582225_110000/LConn3 -- bus48/LConn1
  _CN_142782984_110000_CN_153249112_110000/RConn1 -- T_153249112__/LConn1 -- _CN_153249112_110000_CN_25698690_110000/LConn1
  _CN_142782984_110000_CN_153249112_110000/RConn2 -- T_153249112__/LConn2 -- _CN_153249112_110000_CN_25698690_110000/LConn2
  _CN_142782984_110000_CN_153249112_110000/RConn3 -- T_153249112__/LConn3 -- _CN_153249112_110000_CN_25698690_110000/LConn3 -- bus49/LConn1
  _CN_142782984_110000_CN_25698690_110000/RConn1 -- T_25698690__330kV_skirstymo_pastotė/RConn1 -- _CN_135644003_110000_CN_25698690_110000/LConn1 -- _CN_257684865_110000_CN_25698690_110000/LConn1 -- _CN_25698690_110000_CN_151097769_110000/LConn1 -- L_25698690/LConn1 -- _CN_153249112_110000_CN_25698690_110000/RConn1
  _CN_142782984_110000_CN_25698690_110000/RConn2 -- T_25698690__330kV_skirstymo_pastotė/RConn2 -- _CN_135644003_110000_CN_25698690_110000/LConn2 -- _CN_257684865_110000_CN_25698690_110000/LConn2 -- _CN_25698690_110000_CN_151097769_110000/LConn2 -- L_25698690/LConn2 -- _CN_153249112_110000_CN_25698690_110000/RConn2
  _CN_142782984_110000_CN_25698690_110000/RConn3 -- T_25698690__330kV_skirstymo_pastotė/RConn3 -- _CN_135644003_110000_CN_25698690_110000/LConn3 -- _CN_257684865_110000_CN_25698690_110000/LConn3 -- _CN_25698690_110000_CN_151097769_110000/LConn3 -- L_25698690/LConn3 -- bus50/LConn1 -- _CN_153249112_110000_CN_25698690_110000/RConn3
  T_172590095__/LConn1 -- _CN_172590095_110000_CN_172590108_110000/LConn1
  T_172590095__/LConn2 -- _CN_172590095_110000_CN_172590108_110000/LConn2
  _CN_172590095_110000_CN_172590108_110000/LConn3 -- T_172590095__/LConn3 -- bus51/LConn1
  _CN_172590095_110000_CN_172590108_110000/RConn1 -- T_172590108__/LConn1 -- _CN_172590096_110000_CN_172590108_110000/LConn1
  _CN_172590095_110000_CN_172590108_110000/RConn2 -- T_172590108__/LConn2 -- _CN_172590096_110000_CN_172590108_110000/LConn2
  _CN_172590095_110000_CN_172590108_110000/RConn3 -- T_172590108__/LConn3 -- _CN_172590096_110000_CN_172590108_110000/LConn3 -- bus52/LConn1
  _CN_172590096_110000_CN_172590051_110000/RConn1 -- T_172590096__/LConn1 -- _CN_172590096_110000_CN_172590108_110000/RConn1
  _CN_172590096_110000_CN_172590051_110000/RConn2 -- T_172590096__/LConn2 -- _CN_172590096_110000_CN_172590108_110000/RConn2
  _CN_172590096_110000_CN_172590051_110000/RConn3 -- T_172590096__/LConn3 -- _CN_172590096_110000_CN_172590108_110000/RConn3 -- bus53/LConn1
  T_172590097__/LConn1 -- _CN_172590097_110000_CN_172590051_110000/RConn1
  T_172590097__/LConn2 -- _CN_172590097_110000_CN_172590051_110000/RConn2
  _CN_172590097_110000_CN_172590051_110000/RConn3 -- T_172590097__/LConn3 -- bus54/LConn1
  T_173612890__Garliavos_TP/LConn1 -- _CN_172590100_110000_CN_173612890_110000/RConn1
  T_173612890__Garliavos_TP/LConn2 -- _CN_172590100_110000_CN_173612890_110000/RConn2
  _CN_172590100_110000_CN_173612890_110000/RConn3 -- T_173612890__Garliavos_TP/LConn3 -- bus55/LConn1
  _CN_218214432_110000_CN_218216075_110000/LConn1 -- T_218214432__/LConn1 -- _CN_218214432_110000_CN_260552752_110000/LConn1
  _CN_218214432_110000_CN_218216075_110000/LConn2 -- T_218214432__/LConn2 -- _CN_218214432_110000_CN_260552752_110000/LConn2
  _CN_218214432_110000_CN_218216075_110000/LConn3 -- T_218214432__/LConn3 -- _CN_218214432_110000_CN_260552752_110000/LConn3 -- bus56/LConn1
  _CN_218214432_110000_CN_218216075_110000/RConn1 -- T_218216075_110000;35000;10000_/LConn1 -- _CN_150992936_110000_CN_218216075_110000/LConn1 -- _CN_260552752_110000_CN_218216075_110000/LConn1 -- _CN_192764347_110000_CN_218216075_110000/LConn1 -- _CN_192764283_110000_CN_218216075_110000/LConn1
  _CN_218214432_110000_CN_218216075_110000/RConn2 -- T_218216075_110000;35000;10000_/LConn2 -- _CN_150992936_110000_CN_218216075_110000/LConn2 -- _CN_260552752_110000_CN_218216075_110000/LConn2 -- _CN_192764347_110000_CN_218216075_110000/LConn2 -- _CN_192764283_110000_CN_218216075_110000/LConn2
  _CN_218214432_110000_CN_218216075_110000/RConn3 -- T_218216075_110000;35000;10000_/LConn3 -- _CN_150992936_110000_CN_218216075_110000/LConn3 -- _CN_260552752_110000_CN_218216075_110000/LConn3 -- _CN_192764347_110000_CN_218216075_110000/LConn3 -- _CN_192764283_110000_CN_218216075_110000/LConn3 -- bus57/LConn1
  _CN_218214432_110000_CN_260552752_110000/RConn1 -- T_260552752_110000;35000;10000_/LConn1 -- _CN_260552752_110000_CN_218047622_110000/LConn1 -- _CN_260552752_110000_CN_218223016_110000/LConn1 -- _CN_260552752_110000_CN_151783156_110000/LConn1 -- _CN_260552752_110000_CN_218216075_110000/RConn1 -- _CN_260552752_110000_CN_172407405_110000/LConn1 -- _CN_260552752_110000_CN_218223015_110000/LConn1
  _CN_218214432_110000_CN_260552752_110000/RConn2 -- T_260552752_110000;35000;10000_/LConn2 -- _CN_260552752_110000_CN_218047622_110000/LConn2 -- _CN_260552752_110000_CN_218223016_110000/LConn2 -- _CN_260552752_110000_CN_151783156_110000/LConn2 -- _CN_260552752_110000_CN_218216075_110000/RConn2 -- _CN_260552752_110000_CN_172407405_110000/LConn2 -- _CN_260552752_110000_CN_218223015_110000/LConn2
  _CN_218214432_110000_CN_260552752_110000/RConn3 -- T_260552752_110000;35000;10000_/LConn3 -- _CN_260552752_110000_CN_218047622_110000/LConn3 -- _CN_260552752_110000_CN_218223016_110000/LConn3 -- _CN_260552752_110000_CN_151783156_110000/LConn3 -- _CN_260552752_110000_CN_218216075_110000/RConn3 -- _CN_260552752_110000_CN_172407405_110000/LConn3 -- _CN_260552752_110000_CN_218223015_110000/LConn3 -- bus58/LConn1
  _CN_214455329_110000_CN_210619011_110000/LConn1 -- T_214455329__/LConn1 -- _CN_214455329_110000_CN_171809316_110000/RConn1
  _CN_214455329_110000_CN_210619011_110000/LConn2 -- T_214455329__/LConn2 -- _CN_214455329_110000_CN_171809316_110000/RConn2
  _CN_214455329_110000_CN_210619011_110000/LConn3 -- T_214455329__/LConn3 -- _CN_214455329_110000_CN_171809316_110000/RConn3 -- bus59/LConn1
  _CN_214455329_110000_CN_210619011_110000/RConn1 -- T_210619011__/LConn1 -- _CN_210619008_110000_CN_210619011_110000/LConn1 -- _CN_215632387_110000_CN_210619011_110000/LConn1
  _CN_214455329_110000_CN_210619011_110000/RConn2 -- T_210619011__/LConn2 -- _CN_210619008_110000_CN_210619011_110000/LConn2 -- _CN_215632387_110000_CN_210619011_110000/LConn2
  _CN_214455329_110000_CN_210619011_110000/RConn3 -- T_210619011__/LConn3 -- _CN_210619008_110000_CN_210619011_110000/LConn3 -- _CN_215632387_110000_CN_210619011_110000/LConn3 -- bus60/LConn1
  T_280078882__/LConn1 -- _CN_280078882_110000_CN_221105370_110000/LConn1
  T_280078882__/LConn2 -- _CN_280078882_110000_CN_221105370_110000/LConn2
  _CN_280078882_110000_CN_221105370_110000/LConn3 -- T_280078882__/LConn3 -- bus61/LConn1
  _CN_280078882_110000_CN_221105370_110000/RConn1 -- T_221105370__/LConn1 -- _CN_221105370_110000_CN_172394941_110000/RConn1
  _CN_280078882_110000_CN_221105370_110000/RConn2 -- T_221105370__/LConn2 -- _CN_221105370_110000_CN_172394941_110000/RConn2
  _CN_280078882_110000_CN_221105370_110000/RConn3 -- T_221105370__/LConn3 -- _CN_221105370_110000_CN_172394941_110000/RConn3 -- bus62/LConn1
  T_151237667__/LConn1 -- _CN_151237667_110000_CN_134987741_110000/LConn1
  T_151237667__/LConn2 -- _CN_151237667_110000_CN_134987741_110000/LConn2
  _CN_151237667_110000_CN_134987741_110000/LConn3 -- T_151237667__/LConn3 -- bus63/LConn1
  _CN_151237667_110000_CN_134987741_110000/RConn1 -- T_134987741__/LConn1 -- _CN_174045384_110000_CN_134987741_110000/LConn1
  _CN_151237667_110000_CN_134987741_110000/RConn2 -- T_134987741__/LConn2 -- _CN_174045384_110000_CN_134987741_110000/LConn2
  _CN_151237667_110000_CN_134987741_110000/RConn3 -- T_134987741__/LConn3 -- _CN_174045384_110000_CN_134987741_110000/LConn3 -- bus64/LConn1
  _CN_103275559_110000_CN_103275575_110000/RConn1 -- T_103275575__/LConn1 -- _CN_103275575_110000_CN_104774544_110000/LConn1
  _CN_103275559_110000_CN_103275575_110000/RConn2 -- T_103275575__/LConn2 -- _CN_103275575_110000_CN_104774544_110000/LConn2
  _CN_103275559_110000_CN_103275575_110000/RConn3 -- T_103275575__/LConn3 -- _CN_103275575_110000_CN_104774544_110000/LConn3 -- bus65/LConn1
  _CN_150992936_110000_CN_151783148_110000/LConn1 -- T_150992936_110000;35000;fixme_/LConn1 -- _CN_150992936_110000_CN_218216075_110000/RConn1
  _CN_150992936_110000_CN_151783148_110000/LConn2 -- T_150992936_110000;35000;fixme_/LConn2 -- _CN_150992936_110000_CN_218216075_110000/RConn2
  _CN_150992936_110000_CN_151783148_110000/LConn3 -- T_150992936_110000;35000;fixme_/LConn3 -- _CN_150992936_110000_CN_218216075_110000/RConn3 -- bus66/LConn1
  T_151783148_110000;fixme_/LConn1 -- _CN_150992936_110000_CN_151783148_110000/RConn1
  T_151783148_110000;fixme_/LConn2 -- _CN_150992936_110000_CN_151783148_110000/RConn2
  _CN_150992936_110000_CN_151783148_110000/RConn3 -- T_151783148_110000;fixme_/LConn3 -- bus67/LConn1
  _CN_171630121_110000_CN_103554499_110000/RConn1 -- T_103554499__/LConn1 -- _CN_103554499_110000_CN_217391080_110000/LConn1
  _CN_171630121_110000_CN_103554499_110000/RConn2 -- T_103554499__/LConn2 -- _CN_103554499_110000_CN_217391080_110000/LConn2
  _CN_171630121_110000_CN_103554499_110000/RConn3 -- T_103554499__/LConn3 -- _CN_103554499_110000_CN_217391080_110000/LConn3 -- bus68/LConn1
  T_207755730__/LConn1 -- _CN_171630121_110000_CN_207755730_110000/RConn1
  T_207755730__/LConn2 -- _CN_171630121_110000_CN_207755730_110000/RConn2
  _CN_171630121_110000_CN_207755730_110000/RConn3 -- T_207755730__/LConn3 -- bus69/LConn1
  T_207755729__/LConn1 -- _CN_171630121_110000_CN_207755729_110000/RConn1
  T_207755729__/LConn2 -- _CN_171630121_110000_CN_207755729_110000/RConn2
  _CN_171630121_110000_CN_207755729_110000/RConn3 -- T_207755729__/LConn3 -- bus70/LConn1
  _CN_260552752_110000_CN_218047622_110000/RConn1 -- T_218047622__/LConn1 -- _CN_218047622_110000_CN_220989437_110000/LConn1 -- _CN_218047622_110000_CN_173582226_110000/LConn1 -- _CN_218047622_110000_CN_220986987_110000/LConn1
  _CN_260552752_110000_CN_218047622_110000/RConn2 -- T_218047622__/LConn2 -- _CN_218047622_110000_CN_220989437_110000/LConn2 -- _CN_218047622_110000_CN_173582226_110000/LConn2 -- _CN_218047622_110000_CN_220986987_110000/LConn2
  _CN_260552752_110000_CN_218047622_110000/RConn3 -- T_218047622__/LConn3 -- _CN_218047622_110000_CN_220989437_110000/LConn3 -- bus71/LConn1 -- _CN_218047622_110000_CN_173582226_110000/LConn3 -- _CN_218047622_110000_CN_220986987_110000/LConn3
  T_218223016__/LConn1 -- _CN_260552752_110000_CN_218223016_110000/RConn1
  T_218223016__/LConn2 -- _CN_260552752_110000_CN_218223016_110000/RConn2
  _CN_260552752_110000_CN_218223016_110000/RConn3 -- T_218223016__/LConn3 -- bus72/LConn1
  T_151783156__/LConn1 -- _CN_260552752_110000_CN_151783156_110000/RConn1
  T_151783156__/LConn2 -- _CN_260552752_110000_CN_151783156_110000/RConn2
  _CN_260552752_110000_CN_151783156_110000/RConn3 -- T_151783156__/LConn3 -- bus73/LConn1
  T_172407405__/LConn1 -- _CN_260552752_110000_CN_172407405_110000/RConn1
  T_172407405__/LConn2 -- _CN_260552752_110000_CN_172407405_110000/RConn2
  _CN_260552752_110000_CN_172407405_110000/RConn3 -- T_172407405__/LConn3 -- bus74/LConn1
  _CN_260552752_110000_CN_218223015_110000/RConn1 -- T_218223015__/LConn1 -- _CN_171868832_110000_CN_218223015_110000/LConn1
  _CN_260552752_110000_CN_218223015_110000/RConn2 -- T_218223015__/LConn2 -- _CN_171868832_110000_CN_218223015_110000/LConn2
  _CN_260552752_110000_CN_218223015_110000/RConn3 -- T_218223015__/LConn3 -- _CN_171868832_110000_CN_218223015_110000/LConn3 -- bus75/LConn1
  _CN_171406899_110000_CN_175315244_110000/LConn1 -- T_171406899__/LConn1 -- _CN_171406899_110000_CN_172978107_110000/LConn1
  _CN_171406899_110000_CN_175315244_110000/LConn2 -- T_171406899__/LConn2 -- _CN_171406899_110000_CN_172978107_110000/LConn2
  _CN_171406899_110000_CN_175315244_110000/LConn3 -- T_171406899__/LConn3 -- _CN_171406899_110000_CN_172978107_110000/LConn3 -- bus76/LConn1
  _CN_171406899_110000_CN_175315244_110000/RConn1 -- T_175315244__/LConn1 -- _CN_215632387_110000_CN_175315244_110000/LConn1
  _CN_171406899_110000_CN_175315244_110000/RConn2 -- T_175315244__/LConn2 -- _CN_215632387_110000_CN_175315244_110000/LConn2
  _CN_171406899_110000_CN_175315244_110000/RConn3 -- T_175315244__/LConn3 -- _CN_215632387_110000_CN_175315244_110000/LConn3 -- bus77/LConn1
  _CN_171406899_110000_CN_172978107_110000/RConn1 -- T_172978107__/LConn1 -- _CN_210551439_110000_CN_172978107_110000/LConn1
  _CN_171406899_110000_CN_172978107_110000/RConn2 -- T_172978107__/LConn2 -- _CN_210551439_110000_CN_172978107_110000/LConn2
  _CN_171406899_110000_CN_172978107_110000/RConn3 -- T_172978107__/LConn3 -- _CN_210551439_110000_CN_172978107_110000/LConn3 -- bus78/LConn1
  _CN_210619008_110000_CN_257507721_110000/LConn1 -- T_210619008__/LConn1 -- _CN_210619008_110000_CN_210619011_110000/RConn1 -- _CN_210619008_110000_CN_210612962_110000/LConn1 -- _CN_210619008_110000_CN_210609525_110000/LConn1
  _CN_210619008_110000_CN_257507721_110000/LConn2 -- T_210619008__/LConn2 -- _CN_210619008_110000_CN_210619011_110000/RConn2 -- _CN_210619008_110000_CN_210612962_110000/LConn2 -- _CN_210619008_110000_CN_210609525_110000/LConn2
  _CN_210619008_110000_CN_257507721_110000/LConn3 -- T_210619008__/LConn3 -- _CN_210619008_110000_CN_210619011_110000/RConn3 -- bus79/LConn1 -- _CN_210619008_110000_CN_210612962_110000/LConn3 -- _CN_210619008_110000_CN_210609525_110000/LConn3
  T_257507721__/LConn1 -- _CN_210619008_110000_CN_257507721_110000/RConn1
  T_257507721__/LConn2 -- _CN_210619008_110000_CN_257507721_110000/RConn2
  _CN_210619008_110000_CN_257507721_110000/RConn3 -- T_257507721__/LConn3 -- bus80/LConn1
  T_210612962__/LConn1 -- _CN_210619008_110000_CN_210612962_110000/RConn1
  T_210612962__/LConn2 -- _CN_210619008_110000_CN_210612962_110000/RConn2
  _CN_210619008_110000_CN_210612962_110000/RConn3 -- T_210612962__/LConn3 -- bus81/LConn1
  _CN_210619008_110000_CN_210609525_110000/RConn1 -- T_210609525__/LConn1 -- _CN_210609525_110000_CN_217391080_110000/LConn1
  _CN_210619008_110000_CN_210609525_110000/RConn2 -- T_210609525__/LConn2 -- _CN_210609525_110000_CN_217391080_110000/LConn2
  _CN_210619008_110000_CN_210609525_110000/RConn3 -- T_210609525__/LConn3 -- _CN_210609525_110000_CN_217391080_110000/LConn3 -- bus82/LConn1
  _CN_103275575_110000_CN_104774544_110000/RConn1 -- T_104774544__/LConn1 -- _CN_104774536_110000_CN_104774544_110000/LConn1
  _CN_103275575_110000_CN_104774544_110000/RConn2 -- T_104774544__/LConn2 -- _CN_104774536_110000_CN_104774544_110000/LConn2
  _CN_103275575_110000_CN_104774544_110000/RConn3 -- T_104774544__/LConn3 -- _CN_104774536_110000_CN_104774544_110000/LConn3 -- bus83/LConn1
  _CN_171987005_110000_CN_173944057_110000/LConn1 -- T_171987005_330000;110000;fixme_/RConn1 -- _CN_171987005_110000_CN_173944061_110000/LConn1 -- L_171987005/LConn1
  _CN_171987005_110000_CN_173944057_110000/LConn2 -- T_171987005_330000;110000;fixme_/RConn2 -- _CN_171987005_110000_CN_173944061_110000/LConn2 -- L_171987005/LConn2
  _CN_171987005_110000_CN_173944057_110000/LConn3 -- T_171987005_330000;110000;fixme_/RConn3 -- _CN_171987005_110000_CN_173944061_110000/LConn3 -- L_171987005/LConn3 -- bus84/LConn1
  T_173944057__/LConn1 -- _CN_171987005_110000_CN_173944057_110000/RConn1
  T_173944057__/LConn2 -- _CN_171987005_110000_CN_173944057_110000/RConn2
  _CN_171987005_110000_CN_173944057_110000/RConn3 -- T_173944057__/LConn3 -- bus85/LConn1
  _CN_171987005_110000_CN_173944061_110000/RConn1 -- T_173944061__/LConn1 -- _CN_173944045_110000_CN_173944061_110000/LConn1
  _CN_171987005_110000_CN_173944061_110000/RConn2 -- T_173944061__/LConn2 -- _CN_173944045_110000_CN_173944061_110000/LConn2
  _CN_171987005_110000_CN_173944061_110000/RConn3 -- T_173944061__/LConn3 -- _CN_173944045_110000_CN_173944061_110000/LConn3 -- bus86/LConn1
  _CN_171630144_110000_CN_171630156_110000/LConn1 -- T_171630144__/LConn1 -- _CN_171630144_110000_CN_171630149_110000/LConn1 -- _CN_171630144_110000_CN_171630143_110000/LConn1 -- _CN_171630144_110000_CN_192672898_110000/LConn1 -- _CN_171630144_110000_CN_192646598_110000/LConn1 -- _CN_171630144_110000_CN_171630157_110000/LConn1 -- _CN_171630144_110000_CN_103560163_110000/RConn1
  _CN_171630144_110000_CN_171630156_110000/LConn2 -- T_171630144__/LConn2 -- _CN_171630144_110000_CN_171630149_110000/LConn2 -- _CN_171630144_110000_CN_171630143_110000/LConn2 -- _CN_171630144_110000_CN_192672898_110000/LConn2 -- _CN_171630144_110000_CN_192646598_110000/LConn2 -- _CN_171630144_110000_CN_171630157_110000/LConn2 -- _CN_171630144_110000_CN_103560163_110000/RConn2
  _CN_171630144_110000_CN_171630156_110000/LConn3 -- T_171630144__/LConn3 -- _CN_171630144_110000_CN_171630149_110000/LConn3 -- _CN_171630144_110000_CN_171630143_110000/LConn3 -- _CN_171630144_110000_CN_192672898_110000/LConn3 -- _CN_171630144_110000_CN_192646598_110000/LConn3 -- _CN_171630144_110000_CN_171630157_110000/LConn3 -- _CN_171630144_110000_CN_103560163_110000/RConn3 -- bus87/LConn1
  T_171630156__/LConn1 -- _CN_171630144_110000_CN_171630156_110000/RConn1
  T_171630156__/LConn2 -- _CN_171630144_110000_CN_171630156_110000/RConn2
  _CN_171630144_110000_CN_171630156_110000/RConn3 -- T_171630156__/LConn3 -- bus88/LConn1
  T_171630149__/LConn1 -- _CN_171630144_110000_CN_171630149_110000/RConn1
  T_171630149__/LConn2 -- _CN_171630144_110000_CN_171630149_110000/RConn2
  _CN_171630144_110000_CN_171630149_110000/RConn3 -- T_171630149__/LConn3 -- bus89/LConn1
  T_171630143__/LConn1 -- _CN_171630144_110000_CN_171630143_110000/RConn1
  T_171630143__/LConn2 -- _CN_171630144_110000_CN_171630143_110000/RConn2
  _CN_171630144_110000_CN_171630143_110000/RConn3 -- T_171630143__/LConn3 -- bus90/LConn1
  T_192672898__/LConn1 -- _CN_171630144_110000_CN_192672898_110000/RConn1
  T_192672898__/LConn2 -- _CN_171630144_110000_CN_192672898_110000/RConn2
  _CN_171630144_110000_CN_192672898_110000/RConn3 -- T_192672898__/LConn3 -- bus91/LConn1
  T_192646598__/LConn1 -- _CN_171630144_110000_CN_192646598_110000/RConn1
  T_192646598__/LConn2 -- _CN_171630144_110000_CN_192646598_110000/RConn2
  _CN_171630144_110000_CN_192646598_110000/RConn3 -- T_192646598__/LConn3 -- bus92/LConn1
  T_171630157__/LConn1 -- _CN_171630144_110000_CN_171630157_110000/RConn1
  T_171630157__/LConn2 -- _CN_171630144_110000_CN_171630157_110000/RConn2
  _CN_171630144_110000_CN_171630157_110000/RConn3 -- T_171630157__/LConn3 -- bus93/LConn1
  T_105587267__/LConn1 -- _CN_105587267_110000_CN_243085462_110000/LConn1
  T_105587267__/LConn2 -- _CN_105587267_110000_CN_243085462_110000/LConn2
  _CN_105587267_110000_CN_243085462_110000/LConn3 -- T_105587267__/LConn3 -- bus94/LConn1
  T_243085462__/LConn1 -- _CN_105587267_110000_CN_243085462_110000/RConn1
  T_243085462__/LConn2 -- _CN_105587267_110000_CN_243085462_110000/RConn2
  _CN_105587267_110000_CN_243085462_110000/RConn3 -- T_243085462__/LConn3 -- bus95/LConn1
  _CN_171630153_110000_CN_104774536_110000/LConn1 -- T_171630153_110000;fixme_/LConn1 -- _CN_171630153_110000_CN_239589747_110000/LConn1
  _CN_171630153_110000_CN_104774536_110000/LConn2 -- T_171630153_110000;fixme_/LConn2 -- _CN_171630153_110000_CN_239589747_110000/LConn2
  _CN_171630153_110000_CN_104774536_110000/LConn3 -- T_171630153_110000;fixme_/LConn3 -- _CN_171630153_110000_CN_239589747_110000/LConn3 -- bus96/LConn1
  _CN_171630153_110000_CN_104774536_110000/RConn1 -- T_104774536__/LConn1 -- _CN_104774536_110000_CN_104774544_110000/RConn1
  _CN_171630153_110000_CN_104774536_110000/RConn2 -- T_104774536__/LConn2 -- _CN_104774536_110000_CN_104774544_110000/RConn2
  _CN_171630153_110000_CN_104774536_110000/RConn3 -- T_104774536__/LConn3 -- _CN_104774536_110000_CN_104774544_110000/RConn3 -- bus97/LConn1
  _CN_171630153_110000_CN_239589747_110000/RConn1 -- T_239589747_110000;fixme_/LConn1 -- _CN_239589747_110000_CN_194082693_110000/RConn1
  _CN_171630153_110000_CN_239589747_110000/RConn2 -- T_239589747_110000;fixme_/LConn2 -- _CN_239589747_110000_CN_194082693_110000/RConn2
  _CN_171630153_110000_CN_239589747_110000/RConn3 -- T_239589747_110000;fixme_/LConn3 -- _CN_239589747_110000_CN_194082693_110000/RConn3 -- bus98/LConn1
  T_172019117__/LConn1 -- _CN_215671382_110000_CN_172019117_110000/RConn1
  T_172019117__/LConn2 -- _CN_215671382_110000_CN_172019117_110000/RConn2
  _CN_215671382_110000_CN_172019117_110000/RConn3 -- T_172019117__/LConn3 -- bus99/LConn1
  T_172019087__/LConn1 -- _CN_215671382_110000_CN_172019087_110000/RConn1
  T_172019087__/LConn2 -- _CN_215671382_110000_CN_172019087_110000/RConn2
  _CN_215671382_110000_CN_172019087_110000/RConn3 -- T_172019087__/LConn3 -- bus100/LConn1
  _CN_192764347_110000_CN_192764331_110000/LConn1 -- T_192764347_110000;fixme_/LConn1 -- _CN_192764347_110000_CN_218216075_110000/RConn1 -- _CN_192764347_110000_CN_192764337_110000/LConn1
  _CN_192764347_110000_CN_192764331_110000/LConn2 -- T_192764347_110000;fixme_/LConn2 -- _CN_192764347_110000_CN_218216075_110000/RConn2 -- _CN_192764347_110000_CN_192764337_110000/LConn2
  _CN_192764347_110000_CN_192764331_110000/LConn3 -- T_192764347_110000;fixme_/LConn3 -- _CN_192764347_110000_CN_218216075_110000/RConn3 -- _CN_192764347_110000_CN_192764337_110000/LConn3 -- bus101/LConn1
  _CN_192764347_110000_CN_192764331_110000/RConn1 -- T_192764331__/LConn1 -- _CN_192764331_110000_CN_219084048_110000/LConn1 -- _CN_192764331_110000_CN_192764330_110000/LConn1
  _CN_192764347_110000_CN_192764331_110000/RConn2 -- T_192764331__/LConn2 -- _CN_192764331_110000_CN_219084048_110000/LConn2 -- _CN_192764331_110000_CN_192764330_110000/LConn2
  _CN_192764347_110000_CN_192764331_110000/RConn3 -- T_192764331__/LConn3 -- _CN_192764331_110000_CN_219084048_110000/LConn3 -- _CN_192764331_110000_CN_192764330_110000/LConn3 -- bus102/LConn1
  T_192764337_110000;fixme_/LConn1 -- _CN_192764347_110000_CN_192764337_110000/RConn1
  T_192764337_110000;fixme_/LConn2 -- _CN_192764347_110000_CN_192764337_110000/RConn2
  _CN_192764347_110000_CN_192764337_110000/RConn3 -- T_192764337_110000;fixme_/LConn3 -- bus103/LConn1
  _CN_210557029_110000_CN_181769867_110000/LConn1 -- T_210557029_110000;35000;fixme_/LConn1 -- _CN_210557029_110000_CN_173582216_110000/LConn1 -- _CN_210557029_110000_CN_231990061_110000/LConn1
  _CN_210557029_110000_CN_181769867_110000/LConn2 -- T_210557029_110000;35000;fixme_/LConn2 -- _CN_210557029_110000_CN_173582216_110000/LConn2 -- _CN_210557029_110000_CN_231990061_110000/LConn2
  _CN_210557029_110000_CN_181769867_110000/LConn3 -- T_210557029_110000;35000;fixme_/LConn3 -- _CN_210557029_110000_CN_173582216_110000/LConn3 -- _CN_210557029_110000_CN_231990061_110000/LConn3 -- bus104/LConn1
  _CN_210557029_110000_CN_181769867_110000/RConn1 -- T_181769867__/LConn1 -- _CN_181769867_110000_CN_210555392_110000/LConn1
  _CN_210557029_110000_CN_181769867_110000/RConn2 -- T_181769867__/LConn2 -- _CN_181769867_110000_CN_210555392_110000/LConn2
  _CN_210557029_110000_CN_181769867_110000/RConn3 -- T_181769867__/LConn3 -- _CN_181769867_110000_CN_210555392_110000/LConn3 -- bus105/LConn1
  _CN_210557029_110000_CN_173582216_110000/RConn1 -- T_173582216__/LConn1 -- _CN_257169563_110000_CN_173582216_110000/LConn1
  _CN_210557029_110000_CN_173582216_110000/RConn2 -- T_173582216__/LConn2 -- _CN_257169563_110000_CN_173582216_110000/LConn2
  _CN_210557029_110000_CN_173582216_110000/RConn3 -- T_173582216__/LConn3 -- _CN_257169563_110000_CN_173582216_110000/LConn3 -- bus106/LConn1
  _CN_210557029_110000_CN_231990061_110000/RConn1 -- T_231990061__/LConn1 -- _CN_296374470_110000_CN_231990061_110000/LConn1
  _CN_210557029_110000_CN_231990061_110000/RConn2 -- T_231990061__/LConn2 -- _CN_296374470_110000_CN_231990061_110000/LConn2
  _CN_210557029_110000_CN_231990061_110000/RConn3 -- T_231990061__/LConn3 -- _CN_296374470_110000_CN_231990061_110000/LConn3 -- bus107/LConn1
  _CN_192672875_110000_CN_192677018_110000/LConn1 -- T_192672875__/LConn1 -- _CN_192672875_110000_CN_192672905_110000/LConn1 -- _CN_192672875_110000_CN_192672914_110000/LConn1
  _CN_192672875_110000_CN_192677018_110000/LConn2 -- T_192672875__/LConn2 -- _CN_192672875_110000_CN_192672905_110000/LConn2 -- _CN_192672875_110000_CN_192672914_110000/LConn2
  _CN_192672875_110000_CN_192677018_110000/LConn3 -- T_192672875__/LConn3 -- _CN_192672875_110000_CN_192672905_110000/LConn3 -- _CN_192672875_110000_CN_192672914_110000/LConn3 -- bus108/LConn1
  _CN_192672875_110000_CN_192677018_110000/RConn1 -- T_192677018__/LConn1 -- _CN_192677018_110000_CN_210449206_110000/LConn1
  _CN_192672875_110000_CN_192677018_110000/RConn2 -- T_192677018__/LConn2 -- _CN_192677018_110000_CN_210449206_110000/LConn2
  _CN_192672875_110000_CN_192677018_110000/RConn3 -- T_192677018__/LConn3 -- _CN_192677018_110000_CN_210449206_110000/LConn3 -- bus109/LConn1
  T_192672905__/LConn1 -- _CN_192672875_110000_CN_192672905_110000/RConn1
  T_192672905__/LConn2 -- _CN_192672875_110000_CN_192672905_110000/RConn2
  _CN_192672875_110000_CN_192672905_110000/RConn3 -- T_192672905__/LConn3 -- bus110/LConn1
  T_192672914__/LConn1 -- _CN_192672875_110000_CN_192672914_110000/RConn1
  T_192672914__/LConn2 -- _CN_192672875_110000_CN_192672914_110000/RConn2
  _CN_192672875_110000_CN_192672914_110000/RConn3 -- T_192672914__/LConn3 -- bus111/LConn1
  _CN_172178550_110000_CN_172178562_110000/LConn1 -- T_172178550__/LConn1 -- _CN_172178550_110000_CN_172590051_110000/RConn1
  _CN_172178550_110000_CN_172178562_110000/LConn2 -- T_172178550__/LConn2 -- _CN_172178550_110000_CN_172590051_110000/RConn2
  _CN_172178550_110000_CN_172178562_110000/LConn3 -- T_172178550__/LConn3 -- _CN_172178550_110000_CN_172590051_110000/RConn3 -- bus112/LConn1
  _CN_172178550_110000_CN_172178562_110000/RConn1 -- T_172178562__/LConn1 -- _CN_172178551_110000_CN_172178562_110000/LConn1
  _CN_172178550_110000_CN_172178562_110000/RConn2 -- T_172178562__/LConn2 -- _CN_172178551_110000_CN_172178562_110000/LConn2
  _CN_172178550_110000_CN_172178562_110000/RConn3 -- T_172178562__/LConn3 -- _CN_172178551_110000_CN_172178562_110000/LConn3 -- bus113/LConn1
  _CN_172178551_110000_CN_172178560_110000/LConn1 -- T_172178551__/LConn1 -- _CN_172178551_110000_CN_172178563_110000/LConn1 -- _CN_172178551_110000_CN_172178562_110000/RConn1
  _CN_172178551_110000_CN_172178560_110000/LConn2 -- T_172178551__/LConn2 -- _CN_172178551_110000_CN_172178563_110000/LConn2 -- _CN_172178551_110000_CN_172178562_110000/RConn2
  _CN_172178551_110000_CN_172178560_110000/LConn3 -- T_172178551__/LConn3 -- _CN_172178551_110000_CN_172178563_110000/LConn3 -- bus114/LConn1 -- _CN_172178551_110000_CN_172178562_110000/RConn3
  T_172178560__/LConn1 -- _CN_172178551_110000_CN_172178560_110000/RConn1
  T_172178560__/LConn2 -- _CN_172178551_110000_CN_172178560_110000/RConn2
  _CN_172178551_110000_CN_172178560_110000/RConn3 -- T_172178560__/LConn3 -- bus115/LConn1
  _CN_172178551_110000_CN_172178563_110000/RConn1 -- T_172178563__/LConn1 -- _CN_172178563_110000_CN_226292390_110000/LConn1 -- _CN_172178563_110000_CN_172394924_110000/LConn1 -- _CN_172178563_110000_CN_172394893_110000/LConn1
  _CN_172178551_110000_CN_172178563_110000/RConn2 -- T_172178563__/LConn2 -- _CN_172178563_110000_CN_226292390_110000/LConn2 -- _CN_172178563_110000_CN_172394924_110000/LConn2 -- _CN_172178563_110000_CN_172394893_110000/LConn2
  _CN_172178551_110000_CN_172178563_110000/RConn3 -- T_172178563__/LConn3 -- _CN_172178563_110000_CN_226292390_110000/LConn3 -- _CN_172178563_110000_CN_172394924_110000/LConn3 -- _CN_172178563_110000_CN_172394893_110000/LConn3 -- bus116/LConn1
  G_166814917_Kauno_Algirdo_Brazausko_HE/RConn1 -- _CN_172178556_110000_CN_166814917_110000/RConn1
  G_166814917_Kauno_Algirdo_Brazausko_HE/RConn2 -- _CN_172178556_110000_CN_166814917_110000/RConn2
  _CN_172178556_110000_CN_166814917_110000/RConn3 -- G_166814917_Kauno_Algirdo_Brazausko_HE/RConn3 -- bus117/LConn1
  T_226292390__/LConn1 -- _CN_172178563_110000_CN_226292390_110000/RConn1
  T_226292390__/LConn2 -- _CN_172178563_110000_CN_226292390_110000/RConn2
  _CN_172178563_110000_CN_226292390_110000/RConn3 -- T_226292390__/LConn3 -- bus118/LConn1
  T_172394924__/LConn1 -- _CN_172178563_110000_CN_172394924_110000/RConn1
  T_172394924__/LConn2 -- _CN_172178563_110000_CN_172394924_110000/RConn2
  _CN_172178563_110000_CN_172394924_110000/RConn3 -- T_172394924__/LConn3 -- bus119/LConn1
  _CN_172178563_110000_CN_172394893_110000/RConn1 -- T_172394893__/LConn1 -- _CN_158505202_110000_CN_172394893_110000/LConn1
  _CN_172178563_110000_CN_172394893_110000/RConn2 -- T_172394893__/LConn2 -- _CN_158505202_110000_CN_172394893_110000/LConn2
  _CN_172178563_110000_CN_172394893_110000/RConn3 -- T_172394893__/LConn3 -- _CN_158505202_110000_CN_172394893_110000/LConn3 -- bus120/LConn1
  T_220986987__/LConn1 -- _CN_218047622_110000_CN_220986987_110000/RConn1
  T_220986987__/LConn2 -- _CN_218047622_110000_CN_220986987_110000/RConn2
  _CN_218047622_110000_CN_220986987_110000/RConn3 -- T_220986987__/LConn3 -- bus121/LConn1
  _CN_218047622_110000_CN_173582226_110000/RConn1 -- T_173582226__/LConn1 -- _CN_173582226_110000_CN_173582215_110000/LConn1
  _CN_218047622_110000_CN_173582226_110000/RConn2 -- T_173582226__/LConn2 -- _CN_173582226_110000_CN_173582215_110000/LConn2
  _CN_218047622_110000_CN_173582226_110000/RConn3 -- T_173582226__/LConn3 -- _CN_173582226_110000_CN_173582215_110000/LConn3 -- bus122/LConn1
  T_220989437__/LConn1 -- _CN_218047622_110000_CN_220989437_110000/RConn1
  T_220989437__/LConn2 -- _CN_218047622_110000_CN_220989437_110000/RConn2
  _CN_218047622_110000_CN_220989437_110000/RConn3 -- T_220989437__/LConn3 -- bus123/LConn1
  _CN_127212679_110000_CN_130577811_110000/LConn1 -- T_127212679__Noreikiškių_TP/LConn1 -- _CN_127212679_110000_CN_172019115_110000/LConn1
  _CN_127212679_110000_CN_130577811_110000/LConn2 -- T_127212679__Noreikiškių_TP/LConn2 -- _CN_127212679_110000_CN_172019115_110000/LConn2
  _CN_127212679_110000_CN_130577811_110000/LConn3 -- T_127212679__Noreikiškių_TP/LConn3 -- _CN_127212679_110000_CN_172019115_110000/LConn3 -- bus124/LConn1
  _CN_127212679_110000_CN_130577811_110000/RConn1 -- T_130577811__Vilijampolės_TP/LConn1 -- _CN_88726161_110000_CN_130577811_110000/LConn1
  _CN_127212679_110000_CN_130577811_110000/RConn2 -- T_130577811__Vilijampolės_TP/LConn2 -- _CN_88726161_110000_CN_130577811_110000/LConn2
  _CN_127212679_110000_CN_130577811_110000/RConn3 -- T_130577811__Vilijampolės_TP/LConn3 -- _CN_88726161_110000_CN_130577811_110000/LConn3 -- bus125/LConn1
  T_172019115__Aleksoto_TP/LConn1 -- _CN_127212679_110000_CN_172019115_110000/RConn1
  T_172019115__Aleksoto_TP/LConn2 -- _CN_127212679_110000_CN_172019115_110000/RConn2
  _CN_127212679_110000_CN_172019115_110000/RConn3 -- T_172019115__Aleksoto_TP/LConn3 -- bus126/LConn1
  _CN_181769867_110000_CN_210555392_110000/RConn1 -- T_210555392_110000;35000;fixme_/LConn1 -- _CN_210555392_110000_CN_192764327_110000/LConn1
  _CN_181769867_110000_CN_210555392_110000/RConn2 -- T_210555392_110000;35000;fixme_/LConn2 -- _CN_210555392_110000_CN_192764327_110000/LConn2
  _CN_181769867_110000_CN_210555392_110000/RConn3 -- T_210555392_110000;35000;fixme_/LConn3 -- _CN_210555392_110000_CN_192764327_110000/LConn3 -- bus127/LConn1
  _CN_210551439_110000_CN_172978107_110000/RConn1 -- T_210551439__/LConn1 -- _CN_210551439_110000_CN_210550993_110000/LConn1
  _CN_210551439_110000_CN_172978107_110000/RConn2 -- T_210551439__/LConn2 -- _CN_210551439_110000_CN_210550993_110000/LConn2
  _CN_210551439_110000_CN_172978107_110000/RConn3 -- T_210551439__/LConn3 -- _CN_210551439_110000_CN_210550993_110000/LConn3 -- bus128/LConn1
  _CN_210551439_110000_CN_210550993_110000/RConn1 -- T_210550993__/LConn1 -- _CN_210550993_110000_CN_171406897_110000/LConn1
  _CN_210551439_110000_CN_210550993_110000/RConn2 -- T_210550993__/LConn2 -- _CN_210550993_110000_CN_171406897_110000/LConn2
  _CN_210551439_110000_CN_210550993_110000/RConn3 -- T_210550993__/LConn3 -- _CN_210550993_110000_CN_171406897_110000/LConn3 -- bus129/LConn1
  _CN_88726161_110000_CN_257169562_110000/RConn1 -- T_88726161__Eigulių_TP/LConn1 -- _CN_88726161_110000_CN_130577811_110000/RConn1 -- _CN_88726161_110000_CN_173593029_110000/LConn1 -- _CN_88726161_110000_CN_130577812_110000/LConn1
  _CN_88726161_110000_CN_257169562_110000/RConn2 -- T_88726161__Eigulių_TP/LConn2 -- _CN_88726161_110000_CN_130577811_110000/RConn2 -- _CN_88726161_110000_CN_173593029_110000/LConn2 -- _CN_88726161_110000_CN_130577812_110000/LConn2
  _CN_88726161_110000_CN_257169562_110000/RConn3 -- T_88726161__Eigulių_TP/LConn3 -- _CN_88726161_110000_CN_130577811_110000/RConn3 -- _CN_88726161_110000_CN_173593029_110000/LConn3 -- bus130/LConn1 -- _CN_88726161_110000_CN_130577812_110000/LConn3
  T_130577812__Šilainių_TP/LConn1 -- _CN_88726161_110000_CN_130577812_110000/RConn1
  T_130577812__Šilainių_TP/LConn2 -- _CN_88726161_110000_CN_130577812_110000/RConn2
  _CN_88726161_110000_CN_130577812_110000/RConn3 -- T_130577812__Šilainių_TP/LConn3 -- bus131/LConn1
  T_173593029__Šilko_TP/LConn1 -- _CN_88726161_110000_CN_173593029_110000/RConn1
  T_173593029__Šilko_TP/LConn2 -- _CN_88726161_110000_CN_173593029_110000/RConn2
  _CN_88726161_110000_CN_173593029_110000/RConn3 -- T_173593029__Šilko_TP/LConn3 -- bus132/LConn1
  _CN_210555392_110000_CN_192764327_110000/RConn1 -- T_192764327__/LConn1 -- _CN_192764327_110000_CN_192764330_110000/LConn1
  _CN_210555392_110000_CN_192764327_110000/RConn2 -- T_192764327__/LConn2 -- _CN_192764327_110000_CN_192764330_110000/LConn2
  _CN_210555392_110000_CN_192764327_110000/RConn3 -- T_192764327__/LConn3 -- _CN_192764327_110000_CN_192764330_110000/LConn3 -- bus133/LConn1
  _CN_192677018_110000_CN_210449206_110000/RConn1 -- T_210449206__/LConn1 -- _CN_171229484_110000_CN_210449206_110000/LConn1
  _CN_192677018_110000_CN_210449206_110000/RConn2 -- T_210449206__/LConn2 -- _CN_171229484_110000_CN_210449206_110000/LConn2
  _CN_192677018_110000_CN_210449206_110000/RConn3 -- T_210449206__/LConn3 -- _CN_171229484_110000_CN_210449206_110000/LConn3 -- bus134/LConn1
  _CN_257169563_110000_CN_173582216_110000/RConn1 -- T_257169563__/RConn1 -- L_257169563/LConn1
  _CN_257169563_110000_CN_173582216_110000/RConn2 -- T_257169563__/RConn2 -- L_257169563/LConn2
  _CN_257169563_110000_CN_173582216_110000/RConn3 -- T_257169563__/RConn3 -- L_257169563/LConn3 -- bus135/LConn1
  _CN_171868832_110000_CN_257169562_110000/RConn1 -- T_171868832__/LConn1 -- _CN_171868832_110000_CN_220065702_110000/LConn1 -- _CN_171868832_110000_CN_218223015_110000/RConn1
  _CN_171868832_110000_CN_257169562_110000/RConn2 -- T_171868832__/LConn2 -- _CN_171868832_110000_CN_220065702_110000/LConn2 -- _CN_171868832_110000_CN_218223015_110000/RConn2
  _CN_171868832_110000_CN_257169562_110000/RConn3 -- T_171868832__/LConn3 -- _CN_171868832_110000_CN_220065702_110000/LConn3 -- _CN_171868832_110000_CN_218223015_110000/RConn3 -- bus136/LConn1
  T_220065702__/LConn1 -- _CN_171868832_110000_CN_220065702_110000/RConn1
  T_220065702__/LConn2 -- _CN_171868832_110000_CN_220065702_110000/RConn2
  _CN_171868832_110000_CN_220065702_110000/RConn3 -- T_220065702__/LConn3 -- bus137/LConn1
  _CN_220915873_110000_CN_173591498_110000/LConn1 -- T_220915873__/LConn1 -- _CN_220915873_110000_CN_173591502_110000/LConn1 -- _CN_220915873_110000_CN_173591500_110000/LConn1 -- _CN_220915873_110000_CN_173582225_110000/RConn1 -- _CN_220915873_110000_CN_173944056_110000/LConn1
  _CN_220915873_110000_CN_173591498_110000/LConn2 -- T_220915873__/LConn2 -- _CN_220915873_110000_CN_173591502_110000/LConn2 -- _CN_220915873_110000_CN_173591500_110000/LConn2 -- _CN_220915873_110000_CN_173582225_110000/RConn2 -- _CN_220915873_110000_CN_173944056_110000/LConn2
  _CN_220915873_110000_CN_173591498_110000/LConn3 -- T_220915873__/LConn3 -- _CN_220915873_110000_CN_173591502_110000/LConn3 -- _CN_220915873_110000_CN_173591500_110000/LConn3 -- _CN_220915873_110000_CN_173582225_110000/RConn3 -- bus138/LConn1 -- _CN_220915873_110000_CN_173944056_110000/LConn3
  T_173591498__/LConn1 -- _CN_220915873_110000_CN_173591498_110000/RConn1
  T_173591498__/LConn2 -- _CN_220915873_110000_CN_173591498_110000/RConn2
  _CN_220915873_110000_CN_173591498_110000/RConn3 -- T_173591498__/LConn3 -- bus139/LConn1
  _CN_220915873_110000_CN_173944056_110000/RConn1 -- T_173944056__/LConn1 -- _CN_173944047_110000_CN_173944056_110000/LConn1
  _CN_220915873_110000_CN_173944056_110000/RConn2 -- T_173944056__/LConn2 -- _CN_173944047_110000_CN_173944056_110000/LConn2
  _CN_220915873_110000_CN_173944056_110000/RConn3 -- T_173944056__/LConn3 -- _CN_173944047_110000_CN_173944056_110000/LConn3 -- bus140/LConn1
  T_173591502__/LConn1 -- _CN_220915873_110000_CN_173591502_110000/RConn1
  T_173591502__/LConn2 -- _CN_220915873_110000_CN_173591502_110000/RConn2
  _CN_220915873_110000_CN_173591502_110000/RConn3 -- T_173591502__/LConn3 -- bus141/LConn1
  T_173591500__/LConn1 -- _CN_220915873_110000_CN_173591500_110000/RConn1
  T_173591500__/LConn2 -- _CN_220915873_110000_CN_173591500_110000/RConn2
  _CN_220915873_110000_CN_173591500_110000/RConn3 -- T_173591500__/LConn3 -- bus142/LConn1
  _CN_215632387_110000_CN_175315244_110000/RConn1 -- T_215632387__/LConn1 -- _CN_215632387_110000_CN_171229484_110000/LConn1 -- _CN_215632387_110000_CN_210619011_110000/RConn1 -- _CN_215632387_110000_CN_75909941_110000/LConn1 -- _CN_215632387_110000_CN_99049777_110000/LConn1
  _CN_215632387_110000_CN_175315244_110000/RConn2 -- T_215632387__/LConn2 -- _CN_215632387_110000_CN_171229484_110000/LConn2 -- _CN_215632387_110000_CN_210619011_110000/RConn2 -- _CN_215632387_110000_CN_75909941_110000/LConn2 -- _CN_215632387_110000_CN_99049777_110000/LConn2
  _CN_215632387_110000_CN_175315244_110000/RConn3 -- T_215632387__/LConn3 -- _CN_215632387_110000_CN_171229484_110000/LConn3 -- _CN_215632387_110000_CN_210619011_110000/RConn3 -- _CN_215632387_110000_CN_75909941_110000/LConn3 -- _CN_215632387_110000_CN_99049777_110000/LConn3 -- bus143/LConn1
  _CN_215632387_110000_CN_171229484_110000/RConn1 -- T_171229484__/LConn1 -- _CN_171229484_110000_CN_210457043_110000/LConn1 -- _CN_171229484_110000_CN_210457037_110000/LConn1 -- _CN_171229484_110000_CN_75909941_110000/LConn1 -- _CN_171229484_110000_CN_95066966_110000/LConn1 -- _CN_171229484_110000_CN_210449206_110000/RConn1
  _CN_215632387_110000_CN_171229484_110000/RConn2 -- T_171229484__/LConn2 -- _CN_171229484_110000_CN_210457043_110000/LConn2 -- _CN_171229484_110000_CN_210457037_110000/LConn2 -- _CN_171229484_110000_CN_75909941_110000/LConn2 -- _CN_171229484_110000_CN_95066966_110000/LConn2 -- _CN_171229484_110000_CN_210449206_110000/RConn2
  _CN_215632387_110000_CN_171229484_110000/RConn3 -- T_171229484__/LConn3 -- _CN_171229484_110000_CN_210457043_110000/LConn3 -- _CN_171229484_110000_CN_210457037_110000/LConn3 -- bus144/LConn1 -- _CN_171229484_110000_CN_75909941_110000/LConn3 -- _CN_171229484_110000_CN_95066966_110000/LConn3 -- _CN_171229484_110000_CN_210449206_110000/RConn3
  _CN_215632387_110000_CN_75909941_110000/RConn1 -- T_75909941__Bubių_pastotė/LConn1 -- _CN_171229484_110000_CN_75909941_110000/RConn1
  _CN_215632387_110000_CN_75909941_110000/RConn2 -- T_75909941__Bubių_pastotė/LConn2 -- _CN_171229484_110000_CN_75909941_110000/RConn2
  _CN_215632387_110000_CN_75909941_110000/RConn3 -- T_75909941__Bubių_pastotė/LConn3 -- _CN_171229484_110000_CN_75909941_110000/RConn3 -- bus145/LConn1
  _CN_215632387_110000_CN_99049777_110000/RConn1 -- T_99049777__Gubernijos_pastotė/LConn1 -- _CN_171406897_110000_CN_99049777_110000/LConn1
  _CN_215632387_110000_CN_99049777_110000/RConn2 -- T_99049777__Gubernijos_pastotė/LConn2 -- _CN_171406897_110000_CN_99049777_110000/LConn2
  _CN_215632387_110000_CN_99049777_110000/RConn3 -- T_99049777__Gubernijos_pastotė/LConn3 -- _CN_171406897_110000_CN_99049777_110000/LConn3 -- bus146/LConn1
  _CN_296374470_110000_CN_187242275_110000/LConn1 -- T_296374470__/LConn1 -- _CN_296374470_110000_CN_231990061_110000/RConn1
  _CN_296374470_110000_CN_187242275_110000/LConn2 -- T_296374470__/LConn2 -- _CN_296374470_110000_CN_231990061_110000/RConn2
  _CN_296374470_110000_CN_187242275_110000/LConn3 -- T_296374470__/LConn3 -- _CN_296374470_110000_CN_231990061_110000/RConn3 -- bus147/LConn1
  T_187242275__/LConn1 -- _CN_296374470_110000_CN_187242275_110000/RConn1
  T_187242275__/LConn2 -- _CN_296374470_110000_CN_187242275_110000/RConn2
  _CN_296374470_110000_CN_187242275_110000/RConn3 -- T_187242275__/LConn3 -- bus148/LConn1
  _CN_174045384_110000_CN_134987741_110000/RConn1 -- T_174045384__/LConn1 -- _CN_174045384_110000_CN_158505202_110000/LConn1
  _CN_174045384_110000_CN_134987741_110000/RConn2 -- T_174045384__/LConn2 -- _CN_174045384_110000_CN_158505202_110000/LConn2
  _CN_174045384_110000_CN_134987741_110000/RConn3 -- T_174045384__/LConn3 -- _CN_174045384_110000_CN_158505202_110000/LConn3 -- bus149/LConn1
  _CN_174045384_110000_CN_158505202_110000/RConn1 -- T_158505202__/RConn1 -- _CN_158505202_110000_CN_176323123_110000/LConn1 -- L_158505202/LConn1 -- _CN_158505202_110000_CN_172394893_110000/RConn1 -- _CN_158505202_110000_CN_106172865_110000/LConn1 -- _CN_158505202_110000_CN_192702885_110000/LConn1 -- _CN_158505202_110000_CN_280269221_110000/LConn1
  _CN_174045384_110000_CN_158505202_110000/RConn2 -- T_158505202__/RConn2 -- _CN_158505202_110000_CN_176323123_110000/LConn2 -- L_158505202/LConn2 -- _CN_158505202_110000_CN_172394893_110000/RConn2 -- _CN_158505202_110000_CN_106172865_110000/LConn2 -- _CN_158505202_110000_CN_192702885_110000/LConn2 -- _CN_158505202_110000_CN_280269221_110000/LConn2
  _CN_174045384_110000_CN_158505202_110000/RConn3 -- T_158505202__/RConn3 -- _CN_158505202_110000_CN_176323123_110000/LConn3 -- L_158505202/LConn3 -- bus150/LConn1 -- _CN_158505202_110000_CN_172394893_110000/RConn3 -- _CN_158505202_110000_CN_106172865_110000/LConn3 -- _CN_158505202_110000_CN_192702885_110000/LConn3 -- _CN_158505202_110000_CN_280269221_110000/LConn3
  _CN_210550993_110000_CN_171406897_110000/RConn1 -- T_171406897__/LConn1 -- _CN_171406897_110000_CN_99049777_110000/RConn1 -- _CN_171406897_110000_CN_99049787_110000/LConn1
  _CN_210550993_110000_CN_171406897_110000/RConn2 -- T_171406897__/LConn2 -- _CN_171406897_110000_CN_99049777_110000/RConn2 -- _CN_171406897_110000_CN_99049787_110000/LConn2
  _CN_210550993_110000_CN_171406897_110000/RConn3 -- T_171406897__/LConn3 -- _CN_171406897_110000_CN_99049777_110000/RConn3 -- _CN_171406897_110000_CN_99049787_110000/LConn3 -- bus151/LConn1
  T_219084048__/LConn1 -- _CN_192764331_110000_CN_219084048_110000/RConn1
  T_219084048__/LConn2 -- _CN_192764331_110000_CN_219084048_110000/RConn2
  _CN_192764331_110000_CN_219084048_110000/RConn3 -- T_219084048__/LConn3 -- bus152/LConn1
  _CN_192764331_110000_CN_192764330_110000/RConn1 -- T_192764330__/LConn1 -- _CN_192764327_110000_CN_192764330_110000/RConn1
  _CN_192764331_110000_CN_192764330_110000/RConn2 -- T_192764330__/LConn2 -- _CN_192764327_110000_CN_192764330_110000/RConn2
  _CN_192764331_110000_CN_192764330_110000/RConn3 -- T_192764330__/LConn3 -- _CN_192764327_110000_CN_192764330_110000/RConn3 -- bus153/LConn1
  _CN_192764283_110000_CN_219077432_110000/LConn1 -- T_192764283_330000;110000;fixme_/RConn1 -- _CN_192764283_110000_CN_149815795_110000/LConn1 -- _CN_192764283_110000_CN_149408618_110000/LConn1 -- _CN_192764283_110000_CN_95066982_110000/LConn1 -- _CN_192764283_110000_CN_95866738_110000/LConn1 -- _CN_192764283_110000_CN_218216075_110000/RConn1 -- L_192764283/LConn1
  _CN_192764283_110000_CN_219077432_110000/LConn2 -- T_192764283_330000;110000;fixme_/RConn2 -- _CN_192764283_110000_CN_149815795_110000/LConn2 -- _CN_192764283_110000_CN_149408618_110000/LConn2 -- _CN_192764283_110000_CN_95066982_110000/LConn2 -- _CN_192764283_110000_CN_95866738_110000/LConn2 -- _CN_192764283_110000_CN_218216075_110000/RConn2 -- L_192764283/LConn2
  _CN_192764283_110000_CN_219077432_110000/LConn3 -- T_192764283_330000;110000;fixme_/RConn3 -- _CN_192764283_110000_CN_149815795_110000/LConn3 -- _CN_192764283_110000_CN_149408618_110000/LConn3 -- _CN_192764283_110000_CN_95066982_110000/LConn3 -- _CN_192764283_110000_CN_95866738_110000/LConn3 -- _CN_192764283_110000_CN_218216075_110000/RConn3 -- L_192764283/LConn3 -- bus154/LConn1
  T_219077432_110000;fixme_/LConn1 -- _CN_192764283_110000_CN_219077432_110000/RConn1
  T_219077432_110000;fixme_/LConn2 -- _CN_192764283_110000_CN_219077432_110000/RConn2
  _CN_192764283_110000_CN_219077432_110000/RConn3 -- T_219077432_110000;fixme_/LConn3 -- bus155/LConn1
  T_149815795_110000;35000;fixme_/LConn1 -- _CN_192764283_110000_CN_149815795_110000/RConn1
  T_149815795_110000;35000;fixme_/LConn2 -- _CN_192764283_110000_CN_149815795_110000/RConn2
  _CN_192764283_110000_CN_149815795_110000/RConn3 -- T_149815795_110000;35000;fixme_/LConn3 -- bus156/LConn1
  _CN_192764283_110000_CN_149408618_110000/RConn1 -- T_149408618__/LConn1 -- _CN_95066966_110000_CN_149408618_110000/LConn1
  _CN_192764283_110000_CN_149408618_110000/RConn2 -- T_149408618__/LConn2 -- _CN_95066966_110000_CN_149408618_110000/LConn2
  _CN_192764283_110000_CN_149408618_110000/RConn3 -- T_149408618__/LConn3 -- _CN_95066966_110000_CN_149408618_110000/LConn3 -- bus157/LConn1
  _CN_192764283_110000_CN_95066982_110000/RConn1 -- T_95066982__/LConn1 -- _CN_95066966_110000_CN_95066982_110000/LConn1
  _CN_192764283_110000_CN_95066982_110000/RConn2 -- T_95066982__/LConn2 -- _CN_95066966_110000_CN_95066982_110000/LConn2
  _CN_192764283_110000_CN_95066982_110000/RConn3 -- T_95066982__/LConn3 -- _CN_95066966_110000_CN_95066982_110000/LConn3 -- bus158/LConn1
  T_95866738__/LConn1 -- _CN_192764283_110000_CN_95866738_110000/RConn1
  T_95866738__/LConn2 -- _CN_192764283_110000_CN_95866738_110000/RConn2
  _CN_192764283_110000_CN_95866738_110000/RConn3 -- T_95866738__/LConn3 -- bus159/LConn1
  T_217323242__/LConn1 -- _CN_217323242_110000_CN_192672903_110000/LConn1
  T_217323242__/LConn2 -- _CN_217323242_110000_CN_192672903_110000/LConn2
  _CN_217323242_110000_CN_192672903_110000/LConn3 -- T_217323242__/LConn3 -- bus160/LConn1
  T_192672903__/LConn1 -- _CN_217323242_110000_CN_192672903_110000/RConn1
  T_192672903__/LConn2 -- _CN_217323242_110000_CN_192672903_110000/RConn2
  _CN_217323242_110000_CN_192672903_110000/RConn3 -- T_192672903__/LConn3 -- bus161/LConn1
  _CN_173944045_110000_CN_173944055_110000/LConn1 -- T_173944045__/LConn1 -- _CN_173944045_110000_CN_173944061_110000/RConn1
  _CN_173944045_110000_CN_173944055_110000/LConn2 -- T_173944045__/LConn2 -- _CN_173944045_110000_CN_173944061_110000/RConn2
  _CN_173944045_110000_CN_173944055_110000/LConn3 -- T_173944045__/LConn3 -- _CN_173944045_110000_CN_173944061_110000/RConn3 -- bus162/LConn1
  _CN_173944045_110000_CN_173944055_110000/RConn1 -- T_173944055__/LConn1 -- _CN_173944047_110000_CN_173944055_110000/LConn1
  _CN_173944045_110000_CN_173944055_110000/RConn2 -- T_173944055__/LConn2 -- _CN_173944047_110000_CN_173944055_110000/LConn2
  _CN_173944045_110000_CN_173944055_110000/RConn3 -- T_173944055__/LConn3 -- _CN_173944047_110000_CN_173944055_110000/LConn3 -- bus163/LConn1
  _CN_173944047_110000_CN_173944056_110000/RConn1 -- T_173944047__/LConn1 -- _CN_173944047_110000_CN_173944055_110000/RConn1
  _CN_173944047_110000_CN_173944056_110000/RConn2 -- T_173944047__/LConn2 -- _CN_173944047_110000_CN_173944055_110000/RConn2
  _CN_173944047_110000_CN_173944056_110000/RConn3 -- T_173944047__/LConn3 -- _CN_173944047_110000_CN_173944055_110000/RConn3 -- bus164/LConn1
  T_192702885__/LConn1 -- _CN_158505202_110000_CN_192702885_110000/RConn1
  T_192702885__/LConn2 -- _CN_158505202_110000_CN_192702885_110000/RConn2
  _CN_158505202_110000_CN_192702885_110000/RConn3 -- T_192702885__/LConn3 -- bus165/LConn1
  T_280269221__/LConn1 -- _CN_158505202_110000_CN_280269221_110000/RConn1
  T_280269221__/LConn2 -- _CN_158505202_110000_CN_280269221_110000/RConn2
  _CN_158505202_110000_CN_280269221_110000/RConn3 -- T_280269221__/LConn3 -- bus166/LConn1
  T_106172865__/LConn1 -- _CN_158505202_110000_CN_106172865_110000/RConn1
  T_106172865__/LConn2 -- _CN_158505202_110000_CN_106172865_110000/RConn2
  _CN_158505202_110000_CN_106172865_110000/RConn3 -- T_106172865__/LConn3 -- bus167/LConn1
  T_176323123__/LConn1 -- _CN_158505202_110000_CN_176323123_110000/RConn1
  T_176323123__/LConn2 -- _CN_158505202_110000_CN_176323123_110000/RConn2
  _CN_158505202_110000_CN_176323123_110000/RConn3 -- T_176323123__/LConn3 -- bus168/LConn1
  T_99049787__Zoknių_pastotė/LConn1 -- _CN_171406897_110000_CN_99049787_110000/RConn1
  T_99049787__Zoknių_pastotė/LConn2 -- _CN_171406897_110000_CN_99049787_110000/RConn2
  _CN_171406897_110000_CN_99049787_110000/RConn3 -- T_99049787__Zoknių_pastotė/LConn3 -- bus169/LConn1
  T_172018985__/LConn1 -- _CN_172018985_110000_CN_172019090_110000/RConn1
  T_172018985__/LConn2 -- _CN_172018985_110000_CN_172019090_110000/RConn2
  _CN_172018985_110000_CN_172019090_110000/RConn3 -- T_172018985__/LConn3 -- bus170/LConn1
  _CN_171229484_110000_CN_95066966_110000/RConn1 -- T_95066966__Rėkyvos_pastotė/LConn1 -- _CN_95066966_110000_CN_95066982_110000/RConn1 -- _CN_95066966_110000_CN_149408618_110000/RConn1
  _CN_171229484_110000_CN_95066966_110000/RConn2 -- T_95066966__Rėkyvos_pastotė/LConn2 -- _CN_95066966_110000_CN_95066982_110000/RConn2 -- _CN_95066966_110000_CN_149408618_110000/RConn2
  _CN_171229484_110000_CN_95066966_110000/RConn3 -- T_95066966__Rėkyvos_pastotė/LConn3 -- _CN_95066966_110000_CN_95066982_110000/RConn3 -- _CN_95066966_110000_CN_149408618_110000/RConn3 -- bus171/LConn1
  _CN_171229484_110000_CN_210457043_110000/RConn1 -- T_210457043__/LConn1 -- _CN_210457037_110000_CN_210457043_110000/LConn1
  _CN_171229484_110000_CN_210457043_110000/RConn2 -- T_210457043__/LConn2 -- _CN_210457037_110000_CN_210457043_110000/LConn2
  _CN_171229484_110000_CN_210457043_110000/RConn3 -- T_210457043__/LConn3 -- _CN_210457037_110000_CN_210457043_110000/LConn3 -- bus172/LConn1
  _CN_171229484_110000_CN_210457037_110000/RConn1 -- T_210457037_330000;110000;10000_/LConn1 -- _CN_210457037_110000_CN_210457043_110000/RConn1
  _CN_171229484_110000_CN_210457037_110000/RConn2 -- T_210457037_330000;110000;10000_/LConn2 -- _CN_210457037_110000_CN_210457043_110000/RConn2
  _CN_171229484_110000_CN_210457037_110000/RConn3 -- T_210457037_330000;110000;10000_/LConn3 -- _CN_210457037_110000_CN_210457043_110000/RConn3 -- bus173/LConn1
  _CN_99049810_110000_CN_192764316_110000/LConn1 -- T_99049810_110000;35000;fixme_/LConn1 -- _CN_99049810_110000_CN_192764310_110000/LConn1
  _CN_99049810_110000_CN_192764316_110000/LConn2 -- T_99049810_110000;35000;fixme_/LConn2 -- _CN_99049810_110000_CN_192764310_110000/LConn2
  _CN_99049810_110000_CN_192764316_110000/LConn3 -- T_99049810_110000;35000;fixme_/LConn3 -- _CN_99049810_110000_CN_192764310_110000/LConn3 -- bus174/LConn1
  T_192764316__/LConn1 -- _CN_99049810_110000_CN_192764316_110000/RConn1
  T_192764316__/LConn2 -- _CN_99049810_110000_CN_192764316_110000/RConn2
  _CN_99049810_110000_CN_192764316_110000/RConn3 -- T_192764316__/LConn3 -- bus175/LConn1
  T_192764310__/LConn1 -- _CN_99049810_110000_CN_192764310_110000/RConn1
  T_192764310__/LConn2 -- _CN_99049810_110000_CN_192764310_110000/RConn2
  _CN_99049810_110000_CN_192764310_110000/RConn3 -- T_192764310__/LConn3 -- bus176/LConn1
  _CN_135644003_110000_CN_257684865_110000/LConn1 -- T_135644003__/LConn1 -- _CN_135644003_110000_CN_25698690_110000/RConn1 -- _CN_135644003_110000_CN_257684864_110000/LConn1
  _CN_135644003_110000_CN_257684865_110000/LConn2 -- T_135644003__/LConn2 -- _CN_135644003_110000_CN_25698690_110000/RConn2 -- _CN_135644003_110000_CN_257684864_110000/LConn2
  _CN_135644003_110000_CN_257684865_110000/LConn3 -- T_135644003__/LConn3 -- _CN_135644003_110000_CN_25698690_110000/RConn3 -- _CN_135644003_110000_CN_257684864_110000/LConn3 -- bus177/LConn1
  _CN_135644003_110000_CN_257684865_110000/RConn1 -- T_257684865__/LConn1 -- _CN_257684865_110000_CN_25698690_110000/RConn1
  _CN_135644003_110000_CN_257684865_110000/RConn2 -- T_257684865__/LConn2 -- _CN_257684865_110000_CN_25698690_110000/RConn2
  _CN_135644003_110000_CN_257684865_110000/RConn3 -- T_257684865__/LConn3 -- _CN_257684865_110000_CN_25698690_110000/RConn3 -- bus178/LConn1
  T_257684864__/LConn1 -- _CN_135644003_110000_CN_257684864_110000/RConn1
  T_257684864__/LConn2 -- _CN_135644003_110000_CN_257684864_110000/RConn2
  _CN_135644003_110000_CN_257684864_110000/RConn3 -- T_257684864__/LConn3 -- bus179/LConn1
  T_173582215__/LConn1 -- _CN_173582226_110000_CN_173582215_110000/RConn1
  T_173582215__/LConn2 -- _CN_173582226_110000_CN_173582215_110000/RConn2
  _CN_173582226_110000_CN_173582215_110000/RConn3 -- T_173582215__/LConn3 -- bus180/LConn1
  _CN_210609525_110000_CN_217391080_110000/RConn1 -- T_217391080__/LConn1 -- _CN_103554499_110000_CN_217391080_110000/RConn1
  _CN_210609525_110000_CN_217391080_110000/RConn2 -- T_217391080__/LConn2 -- _CN_103554499_110000_CN_217391080_110000/RConn2
  _CN_210609525_110000_CN_217391080_110000/RConn3 -- T_217391080__/LConn3 -- _CN_103554499_110000_CN_217391080_110000/RConn3 -- bus181/LConn1
  T_151097769__/LConn1 -- _CN_25698690_110000_CN_151097769_110000/RConn1
  T_151097769__/LConn2 -- _CN_25698690_110000_CN_151097769_110000/RConn2
  _CN_25698690_110000_CN_151097769_110000/RConn3 -- T_151097769__/LConn3 -- bus182/LConn1
  T_172445102__/LConn1 -- _CN_172445089_110000_CN_172445102_110000/RConn1
  T_172445102__/LConn2 -- _CN_172445089_110000_CN_172445102_110000/RConn2
  _CN_172445089_110000_CN_172445102_110000/RConn3 -- T_172445102__/LConn3 -- bus183/LConn1
  _CN_172590050_330000_CN_257169562_330000/LConn1 -- T_172590050_330000_/LConn1 -- _CN_172590050_330000_CN_172590115_330000/LConn1 -- _CN_172590050_330000_CN_172589995_330000/LConn1
  _CN_172590050_330000_CN_257169562_330000/LConn2 -- T_172590050_330000_/LConn2 -- _CN_172590050_330000_CN_172590115_330000/LConn2 -- _CN_172590050_330000_CN_172589995_330000/LConn2
  _CN_172590050_330000_CN_257169562_330000/LConn3 -- T_172590050_330000_/LConn3 -- _CN_172590050_330000_CN_172590115_330000/LConn3 -- _CN_172590050_330000_CN_172589995_330000/LConn3 -- bus184/LConn1
  _CN_172590050_330000_CN_257169562_330000/RConn1 -- T_257169562__Kauno_transformatorinė_pastotė/LConn1 -- _CN_258321412_330000_CN_257169562_330000/LConn1
  _CN_172590050_330000_CN_257169562_330000/RConn2 -- T_257169562__Kauno_transformatorinė_pastotė/LConn2 -- _CN_258321412_330000_CN_257169562_330000/LConn2
  _CN_172590050_330000_CN_257169562_330000/RConn3 -- T_257169562__Kauno_transformatorinė_pastotė/LConn3 -- _CN_258321412_330000_CN_257169562_330000/LConn3 -- bus185/LConn1
  T_172590115_330000;110000;fixme_/LConn1 -- _CN_172590050_330000_CN_172590115_330000/RConn1
  T_172590115_330000;110000;fixme_/LConn2 -- _CN_172590050_330000_CN_172590115_330000/RConn2
  _CN_172590050_330000_CN_172590115_330000/RConn3 -- T_172590115_330000;110000;fixme_/LConn3 -- bus186/LConn1
  G_172589995_/RConn1 -- _CN_172590050_330000_CN_172589995_330000/RConn1
  G_172589995_/RConn2 -- _CN_172590050_330000_CN_172589995_330000/RConn2
  _CN_172590050_330000_CN_172589995_330000/RConn3 -- G_172589995_/RConn3 -- bus187/LConn1
  T_25698690__330kV_skirstymo_pastotė/LConn1 -- _CN_25698690_330000_CN_171987005_330000/LConn1
  T_25698690__330kV_skirstymo_pastotė/LConn2 -- _CN_25698690_330000_CN_171987005_330000/LConn2
  _CN_25698690_330000_CN_171987005_330000/LConn3 -- T_25698690__330kV_skirstymo_pastotė/LConn3 -- bus188/LConn1
  _CN_25698690_330000_CN_171987005_330000/RConn1 -- T_171987005_330000;110000;fixme_/LConn1 -- _CN_257169563_330000_CN_171987005_330000/LConn1
  _CN_25698690_330000_CN_171987005_330000/RConn2 -- T_171987005_330000;110000;fixme_/LConn2 -- _CN_257169563_330000_CN_171987005_330000/LConn2
  _CN_25698690_330000_CN_171987005_330000/RConn3 -- T_171987005_330000;110000;fixme_/LConn3 -- _CN_257169563_330000_CN_171987005_330000/LConn3 -- bus189/LConn1
  _CN_172590051_330000_CN_158505202_330000/LConn1 -- T_172590051__/LConn1 -- _CN_172590051_330000_CN_29428018_330000/LConn1
  _CN_172590051_330000_CN_158505202_330000/LConn2 -- T_172590051__/LConn2 -- _CN_172590051_330000_CN_29428018_330000/LConn2
  _CN_172590051_330000_CN_158505202_330000/LConn3 -- T_172590051__/LConn3 -- _CN_172590051_330000_CN_29428018_330000/LConn3 -- bus190/LConn1
  T_158505202__/LConn1 -- _CN_172590051_330000_CN_158505202_330000/RConn1
  T_158505202__/LConn2 -- _CN_172590051_330000_CN_158505202_330000/RConn2
  _CN_172590051_330000_CN_158505202_330000/RConn3 -- T_158505202__/LConn3 -- bus191/LConn1
  T_29428018_330000_ПС_330_кВ_Гродно/LConn1 -- _CN_172590051_330000_CN_29428018_330000/RConn1
  T_29428018_330000_ПС_330_кВ_Гродно/LConn2 -- _CN_172590051_330000_CN_29428018_330000/RConn2
  _CN_172590051_330000_CN_29428018_330000/RConn3 -- T_29428018_330000_ПС_330_кВ_Гродно/LConn3 -- bus192/LConn1
  _CN_258321412_330000_CN_257169562_330000/RConn1 -- T_258321412__/LConn1 -- _CN_258321412_330000_CN_268781050_330000/LConn1
  _CN_258321412_330000_CN_257169562_330000/RConn2 -- T_258321412__/LConn2 -- _CN_258321412_330000_CN_268781050_330000/LConn2
  _CN_258321412_330000_CN_257169562_330000/RConn3 -- T_258321412__/LConn3 -- _CN_258321412_330000_CN_268781050_330000/LConn3 -- bus193/LConn1
  _CN_258321412_330000_CN_268781050_330000/RConn1 -- T_268781050_330000_Bitėnai_Elektros_Tiltas/LConn1 -- _CN_197911127_330000_CN_268781050_330000/LConn1
  _CN_258321412_330000_CN_268781050_330000/RConn2 -- T_268781050_330000_Bitėnai_Elektros_Tiltas/LConn2 -- _CN_197911127_330000_CN_268781050_330000/LConn2
  _CN_258321412_330000_CN_268781050_330000/RConn3 -- T_268781050_330000_Bitėnai_Elektros_Tiltas/LConn3 -- _CN_197911127_330000_CN_268781050_330000/LConn3 -- bus194/LConn1
  _CN_257169563_330000_CN_171987005_330000/RConn1 -- T_257169563__/LConn1 -- _CN_257169563_330000_CN_192764283_330000/LConn1
  _CN_257169563_330000_CN_171987005_330000/RConn2 -- T_257169563__/LConn2 -- _CN_257169563_330000_CN_192764283_330000/LConn2
  _CN_257169563_330000_CN_171987005_330000/RConn3 -- T_257169563__/LConn3 -- _CN_257169563_330000_CN_192764283_330000/LConn3 -- bus195/LConn1
  _CN_257169563_330000_CN_192764283_330000/RConn1 -- T_192764283_330000;110000;fixme_/LConn1 -- _CN_220065689_330000_CN_192764283_330000/LConn1
  _CN_257169563_330000_CN_192764283_330000/RConn2 -- T_192764283_330000;110000;fixme_/LConn2 -- _CN_220065689_330000_CN_192764283_330000/LConn2
  _CN_257169563_330000_CN_192764283_330000/RConn3 -- T_192764283_330000;110000;fixme_/LConn3 -- _CN_220065689_330000_CN_192764283_330000/LConn3 -- bus196/LConn1
  T_197911127_330000;110000;15000;6000_ПС_330_кВ_«Советск»/LConn1 -- _CN_197911127_330000_CN_268781050_330000/RConn1
  T_197911127_330000;110000;15000;6000_ПС_330_кВ_«Советск»/LConn2 -- _CN_197911127_330000_CN_268781050_330000/RConn2
  _CN_197911127_330000_CN_268781050_330000/RConn3 -- T_197911127_330000;110000;15000;6000_ПС_330_кВ_«Советск»/LConn3 -- bus197/LConn1
  T_220065689__/LConn1 -- _CN_220065689_330000_CN_192764283_330000/RConn1
  T_220065689__/LConn2 -- _CN_220065689_330000_CN_192764283_330000/RConn2
  _CN_220065689_330000_CN_192764283_330000/RConn3 -- T_220065689__/LConn3 -- bus198/LConn1
  T_172590080__/RConn1 -- L_172590080/LConn1
  T_172590080__/RConn2 -- L_172590080/LConn2
  L_172590080/LConn3 -- T_172590080__/RConn3 -- bus199/LConn1
  T_172178556__/RConn1 -- L_172178556/LConn1
  T_172178556__/RConn2 -- L_172178556/LConn2
  L_172178556/LConn3 -- T_172178556__/RConn3 -- bus200/LConn1
  T_172590100__Rokų_TP/RConn1 -- L_172590100/LConn1
  T_172590100__Rokų_TP/RConn2 -- L_172590100/LConn2
  L_172590100/LConn3 -- T_172590100__Rokų_TP/RConn3 -- bus201/LConn1
  T_172590098__Drobės_TP/RConn1 -- L_172590098/LConn1
  T_172590098__Drobės_TP/RConn2 -- L_172590098/LConn2
  L_172590098/LConn3 -- T_172590098__Drobės_TP/RConn3 -- bus202/LConn1
  T_135895688__Palemono_Traukos_TP/RConn1 -- L_135895688/LConn1
  T_135895688__Palemono_Traukos_TP/RConn2 -- L_135895688/LConn2
  L_135895688/LConn3 -- T_135895688__Palemono_Traukos_TP/RConn3 -- bus203/LConn1
  T_172590101__Petrašiūnų_TP/RConn1 -- L_172590101/LConn1
  T_172590101__Petrašiūnų_TP/RConn2 -- L_172590101/LConn2
  L_172590101/LConn3 -- T_172590101__Petrašiūnų_TP/RConn3 -- bus204/LConn1
  T_172590105__Ketaus_TP/RConn1 -- L_172590105/LConn1
  T_172590105__Ketaus_TP/RConn2 -- L_172590105/LConn2
  L_172590105/LConn3 -- T_172590105__Ketaus_TP/RConn3 -- bus205/LConn1
  T_173765447__Pluošto_TP/RConn1 -- L_173765447/LConn1
  T_173765447__Pluošto_TP/RConn2 -- L_173765447/LConn2
  L_173765447/LConn3 -- T_173765447__Pluošto_TP/RConn3 -- bus206/LConn1
  T_172590075__Žasmos_TP/RConn1 -- L_172590075/LConn1
  T_172590075__Žasmos_TP/RConn2 -- L_172590075/LConn2
  L_172590075/LConn3 -- T_172590075__Žasmos_TP/RConn3 -- bus207/LConn1
  T_172590076__/RConn1 -- L_172590076/LConn1
  T_172590076__/RConn2 -- L_172590076/LConn2
  L_172590076/LConn3 -- T_172590076__/RConn3 -- bus208/LConn1
  T_172590116__/RConn1 -- L_172590116/LConn1
  T_172590116__/RConn2 -- L_172590116/LConn2
  L_172590116/LConn3 -- T_172590116__/RConn3 -- bus209/LConn1
  T_172445101__/RConn1 -- L_172445101/LConn1
  T_172445101__/RConn2 -- L_172445101/LConn2
  L_172445101/LConn3 -- T_172445101__/RConn3 -- bus210/LConn1
  T_172590088__/RConn1 -- L_172590088/LConn1
  T_172590088__/RConn2 -- L_172590088/LConn2
  L_172590088/LConn3 -- T_172590088__/RConn3 -- bus211/LConn1
  T_265807988__/RConn1 -- L_265807988/LConn1
  T_265807988__/RConn2 -- L_265807988/LConn2
  L_265807988/LConn3 -- T_265807988__/RConn3 -- bus212/LConn1
  T_215671382__/RConn1 -- L_215671382/LConn1
  T_215671382__/RConn2 -- L_215671382/LConn2
  L_215671382/LConn3 -- T_215671382__/RConn3 -- bus213/LConn1
  T_172445107__/RConn1 -- L_172445107/LConn1
  T_172445107__/RConn2 -- L_172445107/LConn2
  L_172445107/LConn3 -- T_172445107__/RConn3 -- bus214/LConn1
  T_172445089__/RConn1 -- L_172445089/LConn1
  T_172445089__/RConn2 -- L_172445089/LConn2
  L_172445089/LConn3 -- T_172445089__/RConn3 -- bus215/LConn1
  T_172445103__/RConn1 -- L_172445103/LConn1
  T_172445103__/RConn2 -- L_172445103/LConn2
  L_172445103/LConn3 -- T_172445103__/RConn3 -- bus216/LConn1
  T_172019127__/RConn1 -- L_172019127/LConn1
  T_172019127__/RConn2 -- L_172019127/LConn2
  L_172019127/LConn3 -- T_172019127__/RConn3 -- bus217/LConn1
  T_172394941__/RConn1 -- L_172394941/LConn1
  T_172394941__/RConn2 -- L_172394941/LConn2
  L_172394941/LConn3 -- T_172394941__/RConn3 -- bus218/LConn1
  T_214227031__/RConn1 -- L_214227031/LConn1
  T_214227031__/RConn2 -- L_214227031/LConn2
  L_214227031/LConn3 -- T_214227031__/RConn3 -- bus219/LConn1
  T_158244489__Palemono_TP/RConn1 -- L_158244489/LConn1
  T_158244489__Palemono_TP/RConn2 -- L_158244489/LConn2
  L_158244489/LConn3 -- T_158244489__Palemono_TP/RConn3 -- bus220/LConn1
  T_172394923__/RConn1 -- L_172394923/LConn1
  T_172394923__/RConn2 -- L_172394923/LConn2
  L_172394923/LConn3 -- T_172394923__/RConn3 -- bus221/LConn1
  T_172590081__/RConn1 -- L_172590081/LConn1
  T_172590081__/RConn2 -- L_172590081/LConn2
  L_172590081/LConn3 -- T_172590081__/RConn3 -- bus222/LConn1
  T_214649882__/RConn1 -- L_214649882/LConn1
  T_214649882__/RConn2 -- L_214649882/LConn2
  L_214649882/LConn3 -- T_214649882__/RConn3 -- bus223/LConn1
  T_172019090__/RConn1 -- L_172019090/LConn1
  T_172019090__/RConn2 -- L_172019090/LConn2
  L_172019090/LConn3 -- T_172019090__/RConn3 -- bus224/LConn1
  T_210995832__/RConn1 -- L_210995832/LConn1
  T_210995832__/RConn2 -- L_210995832/LConn2
  L_210995832/LConn3 -- T_210995832__/RConn3 -- bus225/LConn1
  T_194082693__/RConn1 -- L_194082693/LConn1
  T_194082693__/RConn2 -- L_194082693/LConn2
  L_194082693/LConn3 -- T_194082693__/RConn3 -- bus226/LConn1
  T_212007661_110000;fixme_/RConn1 -- L_212007661/LConn1
  T_212007661_110000;fixme_/RConn2 -- L_212007661/LConn2
  L_212007661/LConn3 -- T_212007661_110000;fixme_/RConn3 -- bus227/LConn1
  T_214674623__/RConn1 -- L_214674623/LConn1
  T_214674623__/RConn2 -- L_214674623/LConn2
  L_214674623/LConn3 -- T_214674623__/RConn3 -- bus228/LConn1
  T_172019085__/RConn1 -- L_172019085/LConn1
  T_172019085__/RConn2 -- L_172019085/LConn2
  L_172019085/LConn3 -- T_172019085__/RConn3 -- bus229/LConn1
